simulink library "mbd_s32k1xx_ec_toolbox"  (Simulink 9.0)
(part 7 of 8)

      mask TypeOptions pinFtmCh5: None | PTD15: [FTM0_CH0 | FTM Channel] | PTB13: [FTM0_CH1 | FTM Channel] | PTC1: [FTM0_CH1 | FTM Channel] | PTD16: [FTM0_CH1 | FTM Channel] | PTC2: [FTM0_CH2 | FTM Channel] | PTD0: [FTM0_CH2 | FTM Channel] | PTC3: [FTM0_CH3 | FTM Channel] | PTD1: [FTM0_CH3 | FTM Channel] | PTB4: [FTM0_CH4 | FTM Channel] | PTB5: [FTM0_CH5 | FTM Channel] | PTE8: [FTM0_CH6 | FTM Channel] | PTE9: [FTM0_CH7 | FTM Channel] | PTB2: [FTM1_CH0 | FTM Channel] | PTC4: [FTM1_CH0 | FTM Channel] | PTA1: [FTM1_CH1 | FTM Channel] | PTB3: [FTM1_CH1 | FTM Channel] | PTC14: [FTM1_CH2 | FTM Channel] | PTC15: [FTM1_CH3 | FTM Channel] | PTA10: [FTM1_CH4 | FTM Channel] | PTA11: [FTM1_CH5 | FTM Channel] | PTA12: [FTM1_CH6 | FTM Channel] | PTA13: [FTM1_CH7 | FTM Channel] | PTC1: [FTM1_CH7 | FTM Channel] | PTD15: [FTM0_CH0 | FTM Channel] | PTB13: [FTM0_CH1 | FTM Channel] | PTC1: [FTM0_CH1 | FTM Channel] | PTD16: [FTM0_CH1 | FTM Channel] | PTC2: [FTM0_CH2 | FTM Channel] | PTD0: [FTM0_CH2 | FTM Channel] | PTC3: [FTM0_CH3 | FTM Channel] | PTD1: [FTM0_CH3 | FTM Channel] | PTB4: [FTM0_CH4 | FTM Channel] | PTB5: [FTM0_CH5 | FTM Channel] | PTE8: [FTM0_CH6 | FTM Channel] | PTE9: [FTM0_CH7 | FTM Channel] | PTB2: [FTM1_CH0 | FTM Channel] | PTC4: [FTM1_CH0 | FTM Channel] | PTA1: [FTM1_CH1 | FTM Channel] | PTB3: [FTM1_CH1 | FTM Channel] | PTC14: [FTM1_CH2 | FTM Channel] | PTC15: [FTM1_CH3 | FTM Channel] | PTA10: [FTM1_CH4 | FTM Channel] | PTA11: [FTM1_CH5 | FTM Channel] | PTA12: [FTM1_CH6 | FTM Channel] | PTA13: [FTM1_CH7 | FTM Channel] | PTC1: [FTM1_CH7 | FTM Channel] | PTD15: [FTM0_CH0 | FTM Channel] | PTB13: [FTM0_CH1 | FTM Channel] | PTC1: [FTM0_CH1 | FTM Channel] | PTD16: [FTM0_CH1 | FTM Channel] | PTC2: [FTM0_CH2 | FTM Channel] | PTD0: [FTM0_CH2 | FTM Channel] | PTC3: [FTM0_CH3 | FTM Channel] | PTD1: [FTM0_CH3 | FTM Channel] | PTB4: [FTM0_CH4 | FTM Channel] | PTB5: [FTM0_CH5 | FTM Channel] | PTE8: [FTM0_CH6 | FTM Channel] | PTE9: [FTM0_CH7 | FTM Channel] | PTB2: [FTM1_CH0 | FTM Channel] | PTC4: [FTM1_CH0 | FTM Channel] | PTA1: [FTM1_CH1 | FTM Channel] | PTB3: [FTM1_CH1 | FTM Channel] | PTC14: [FTM1_CH2 | FTM Channel] | PTC15: [FTM1_CH3 | FTM Channel] | PTA10: [FTM1_CH4 | FTM Channel] | PTA11: [FTM1_CH5 | FTM Channel] | PTA12: [FTM1_CH6 | FTM Channel] | PTA13: [FTM1_CH7 | FTM Channel] | PTC1: [FTM1_CH7 | FTM Channel] | PTC5: [FTM2_CH0 | FTM Channel] | PTD0: [FTM2_CH0 | FTM Channel] | PTD10: [FTM2_CH0 | FTM Channel] | PTA0: [FTM2_CH1 | FTM Channel] | PTD1: [FTM2_CH1 | FTM Channel] | PTD11: [FTM2_CH1 | FTM Channel] | PTD12: [FTM2_CH2 | FTM Channel] | PTE4: [FTM2_CH2 | FTM Channel] | PTD5: [FTM2_CH3 | FTM Channel] | PTE5: [FTM2_CH3 | FTM Channel] | PTD13: [FTM2_CH4 | FTM Channel] | PTE10: [FTM2_CH4 | FTM Channel] | PTD14: [FTM2_CH5 | FTM Channel] | PTE11: [FTM2_CH5 | FTM Channel] | PTC12: [FTM2_CH6 | FTM Channel] | PTE15: [FTM2_CH6 | FTM Channel] | PTC13: [FTM2_CH7 | FTM Channel] | PTE16: [FTM2_CH7 | FTM Channel] | PTA2: [FTM3_CH0 | FTM Channel] | PTB8: [FTM3_CH0 | FTM Channel] | PTA3: [FTM3_CH1 | FTM Channel] | PTB9: [FTM3_CH1 | FTM Channel] | PTB10: [FTM3_CH2 | FTM Channel] | PTC6: [FTM3_CH2 | FTM Channel] | PTB11: [FTM3_CH3 | FTM Channel] | PTC7: [FTM3_CH3 | FTM Channel] | PTC10: [FTM3_CH4 | FTM Channel] | PTD2: [FTM3_CH4 | FTM Channel] | PTC11: [FTM3_CH5 | FTM Channel] | PTD3: [FTM3_CH5 | FTM Channel] | PTC12: [FTM3_CH6 | FTM Channel] | PTE2: [FTM3_CH6 | FTM Channel] | PTC13: [FTM3_CH7 | FTM Channel] | PTE6: [FTM3_CH7 | FTM Channel] | PTD15: [FTM0_CH0 | FTM Channel] | PTB13: [FTM0_CH1 | FTM Channel] | PTC1: [FTM0_CH1 | FTM Channel] | PTD16: [FTM0_CH1 | FTM Channel] | PTC2: [FTM0_CH2 | FTM Channel] | PTD0: [FTM0_CH2 | FTM Channel] | PTC3: [FTM0_CH3 | FTM Channel] | PTD1: [FTM0_CH3 | FTM Channel] | PTB4: [FTM0_CH4 | FTM Channel] | PTB5: [FTM0_CH5 | FTM Channel] | PTE8: [FTM0_CH6 | FTM Channel] | PTE9: [FTM0_CH7 | FTM Channel] | PTB2: [FTM1_CH0 | FTM Channel] | PTC4: [FTM1_CH0 | FTM Channel] | PTA1: [FTM1_CH1 | FTM Channel] | PTB3: [FTM1_CH1 | FTM Channel] | PTC14: [FTM1_CH2 | FTM Channel] | PTC15: [FTM1_CH3 | FTM Channel] | PTA10: [FTM1_CH4 | FTM Channel] | PTA11: [FTM1_CH5 | FTM Channel] | PTA12: [FTM1_CH6 | FTM Channel] | PTA13: [FTM1_CH7 | FTM Channel] | PTC1: [FTM1_CH7 | FTM Channel] | PTC5: [FTM2_CH0 | FTM Channel] | PTD0: [FTM2_CH0 | FTM Channel] | PTD10: [FTM2_CH0 | FTM Channel] | PTA0: [FTM2_CH1 | FTM Channel] | PTD1: [FTM2_CH1 | FTM Channel] | PTD11: [FTM2_CH1 | FTM Channel] | PTD12: [FTM2_CH2 | FTM Channel] | PTE4: [FTM2_CH2 | FTM Channel] | PTD5: [FTM2_CH3 | FTM Channel] | PTE5: [FTM2_CH3 | FTM Channel] | PTD13: [FTM2_CH4 | FTM Channel] | PTE10: [FTM2_CH4 | FTM Channel] | PTD14: [FTM2_CH5 | FTM Channel] | PTE11: [FTM2_CH5 | FTM Channel] | PTC12: [FTM2_CH6 | FTM Channel] | PTE15: [FTM2_CH6 | FTM Channel] | PTC13: [FTM2_CH7 | FTM Channel] | PTE16: [FTM2_CH7 | FTM Channel] | PTA2: [FTM3_CH0 | FTM Channel] | PTB8: [FTM3_CH0 | FTM Channel] | PTA3: [FTM3_CH1 | FTM Channel] | PTB9: [FTM3_CH1 | FTM Channel] | PTB10: [FTM3_CH2 | FTM Channel] | PTC6: [FTM3_CH2 | FTM Channel] | PTB11: [FTM3_CH3 | FTM Channel] | PTC7: [FTM3_CH3 | FTM Channel] | PTC10: [FTM3_CH4 | FTM Channel] | PTD2: [FTM3_CH4 | FTM Channel] | PTC11: [FTM3_CH5 | FTM Channel] | PTD3: [FTM3_CH5 | FTM Channel] | PTC12: [FTM3_CH6 | FTM Channel] | PTE2: [FTM3_CH6 | FTM Channel] | PTC13: [FTM3_CH7 | FTM Channel] | PTE6: [FTM3_CH7 | FTM Channel] | PTD15: [FTM0_CH0 | FTM Channel] | PTB13: [FTM0_CH1 | FTM Channel] | PTC1: [FTM0_CH1 | FTM Channel] | PTD16: [FTM0_CH1 | FTM Channel] | PTC2: [FTM0_CH2 | FTM Channel] | PTD0: [FTM0_CH2 | FTM Channel] | PTC3: [FTM0_CH3 | FTM Channel] | PTD1: [FTM0_CH3 | FTM Channel] | PTB4: [FTM0_CH4 | FTM Channel] | PTB5: [FTM0_CH5 | FTM Channel] | PTE8: [FTM0_CH6 | FTM Channel] | PTE9: [FTM0_CH7 | FTM Channel] | PTB2: [FTM1_CH0 | FTM Channel] | PTC4: [FTM1_CH0 | FTM Channel] | PTA1: [FTM1_CH1 | FTM Channel] | PTB3: [FTM1_CH1 | FTM Channel] | PTC14: [FTM1_CH2 | FTM Channel] | PTC15: [FTM1_CH3 | FTM Channel] | PTA10: [FTM1_CH4 | FTM Channel] | PTA11: [FTM1_CH5 | FTM Channel] | PTA12: [FTM1_CH6 | FTM Channel] | PTA13: [FTM1_CH7 | FTM Channel] | PTC1: [FTM1_CH7 | FTM Channel] | PTC5: [FTM2_CH0 | FTM Channel] | PTD0: [FTM2_CH0 | FTM Channel] | PTD10: [FTM2_CH0 | FTM Channel] | PTA0: [FTM2_CH1 | FTM Channel] | PTD1: [FTM2_CH1 | FTM Channel] | PTD11: [FTM2_CH1 | FTM Channel] | PTD12: [FTM2_CH2 | FTM Channel] | PTE4: [FTM2_CH2 | FTM Channel] | PTD5: [FTM2_CH3 | FTM Channel] | PTE5: [FTM2_CH3 | FTM Channel] | PTD13: [FTM2_CH4 | FTM Channel] | PTE10: [FTM2_CH4 | FTM Channel] | PTD14: [FTM2_CH5 | FTM Channel] | PTE11: [FTM2_CH5 | FTM Channel] | PTC12: [FTM2_CH6 | FTM Channel] | PTE15: [FTM2_CH6 | FTM Channel] | PTC13: [FTM2_CH7 | FTM Channel] | PTE16: [FTM2_CH7 | FTM Channel] | PTA2: [FTM3_CH0 | FTM Channel] | PTB8: [FTM3_CH0 | FTM Channel] | PTA3: [FTM3_CH1 | FTM Channel] | PTB9: [FTM3_CH1 | FTM Channel] | PTB10: [FTM3_CH2 | FTM Channel] | PTC6: [FTM3_CH2 | FTM Channel] | PTB11: [FTM3_CH3 | FTM Channel] | PTC7: [FTM3_CH3 | FTM Channel] | PTC10: [FTM3_CH4 | FTM Channel] | PTD2: [FTM3_CH4 | FTM Channel] | PTC11: [FTM3_CH5 | FTM Channel] | PTD3: [FTM3_CH5 | FTM Channel] | PTC12: [FTM3_CH6 | FTM Channel] | PTE2: [FTM3_CH6 | FTM Channel] | PTC13: [FTM3_CH7 | FTM Channel] | PTE6: [FTM3_CH7 | FTM Channel] | PTE20: [FTM4_CH0 | FTM Channel] | PTE21: [FTM4_CH1 | FTM Channel] | PTC11: [FTM4_CH2 | FTM Channel] | PTE22: [FTM4_CH2 | FTM Channel] | PTE23: [FTM4_CH3 | FTM Channel] | PTC27: [FTM4_CH4 | FTM Channel] | PTE24: [FTM4_CH4 | FTM Channel] | PTB1: [FTM4_CH5 | FTM Channel] | PTE13: [FTM4_CH5 | FTM Channel] | PTE25: [FTM4_CH5 | FTM Channel] | PTB0: [FTM4_CH6 | FTM Channel] | PTC28: [FTM4_CH7 | FTM Channel] | PTA25: [FTM5_CH0 | FTM Channel] | PTC9: [FTM5_CH0 | FTM Channel] | PTA26: [FTM5_CH1 | FTM Channel] | PTC8: [FTM5_CH1 | FTM Channel] | PTA27: [FTM5_CH2 | FTM Channel] | PTC29: [FTM5_CH2 | FTM Channel] | PTA7: [FTM5_CH3 | FTM Channel] | PTA28: [FTM5_CH3 | FTM Channel] | PTA29: [FTM5_CH4 | FTM Channel] | PTC30: [FTM5_CH4 | FTM Channel] | PTA6: [FTM5_CH5 | FTM Channel] | PTA30: [FTM5_CH5 | FTM Channel] | PTA31: [FTM5_CH6 | FTM Channel] | PTC31: [FTM5_CH6 | FTM Channel] | PTB18: [FTM5_CH7 | FTM Channel] | PTD18: [FTM5_CH7 | FTM Channel] | PTD15: [FTM0_CH0 | FTM Channel] | PTB13: [FTM0_CH1 | FTM Channel] | PTC1: [FTM0_CH1 | FTM Channel] | PTD16: [FTM0_CH1 | FTM Channel] | PTC2: [FTM0_CH2 | FTM Channel] | PTD0: [FTM0_CH2 | FTM Channel] | PTC3: [FTM0_CH3 | FTM Channel] | PTD1: [FTM0_CH3 | FTM Channel] | PTB4: [FTM0_CH4 | FTM Channel] | PTB5: [FTM0_CH5 | FTM Channel] | PTE8: [FTM0_CH6 | FTM Channel] | PTE9: [FTM0_CH7 | FTM Channel] | PTB2: [FTM1_CH0 | FTM Channel] | PTC4: [FTM1_CH0 | FTM Channel] | PTA1: [FTM1_CH1 | FTM Channel] | PTB3: [FTM1_CH1 | FTM Channel] | PTC14: [FTM1_CH2 | FTM Channel] | PTC15: [FTM1_CH3 | FTM Channel] | PTA10: [FTM1_CH4 | FTM Channel] | PTA11: [FTM1_CH5 | FTM Channel] | PTA12: [FTM1_CH6 | FTM Channel] | PTA13: [FTM1_CH7 | FTM Channel] | PTC1: [FTM1_CH7 | FTM Channel] | PTC5: [FTM2_CH0 | FTM Channel] | PTD0: [FTM2_CH0 | FTM Channel] | PTD10: [FTM2_CH0 | FTM Channel] | PTA0: [FTM2_CH1 | FTM Channel] | PTD1: [FTM2_CH1 | FTM Channel] | PTD11: [FTM2_CH1 | FTM Channel] | PTD12: [FTM2_CH2 | FTM Channel] | PTE4: [FTM2_CH2 | FTM Channel] | PTD5: [FTM2_CH3 | FTM Channel] | PTE5: [FTM2_CH3 | FTM Channel] | PTD13: [FTM2_CH4 | FTM Channel] | PTE10: [FTM2_CH4 | FTM Channel] | PTD14: [FTM2_CH5 | FTM Channel] | PTE11: [FTM2_CH5 | FTM Channel] | PTC12: [FTM2_CH6 | FTM Channel] | PTE15: [FTM2_CH6 | FTM Channel] | PTC13: [FTM2_CH7 | FTM Channel] | PTE16: [FTM2_CH7 | FTM Channel] | PTA2: [FTM3_CH0 | FTM Channel] | PTB8: [FTM3_CH0 | FTM Channel] | PTA3: [FTM3_CH1 | FTM Channel] | PTB9: [FTM3_CH1 | FTM Channel] | PTB10: [FTM3_CH2 | FTM Channel] | PTC6: [FTM3_CH2 | FTM Channel] | PTB11: [FTM3_CH3 | FTM Channel] | PTC7: [FTM3_CH3 | FTM Channel] | PTC10: [FTM3_CH4 | FTM Channel] | PTD2: [FTM3_CH4 | FTM Channel] | PTC11: [FTM3_CH5 | FTM Channel] | PTD3: [FTM3_CH5 | FTM Channel] | PTC12: [FTM3_CH6 | FTM Channel] | PTE2: [FTM3_CH6 | FTM Channel] | PTC13: [FTM3_CH7 | FTM Channel] | PTE6: [FTM3_CH7 | FTM Channel] | PTE20: [FTM4_CH0 | FTM Channel] | PTE21: [FTM4_CH1 | FTM Channel] | PTC11: [FTM4_CH2 | FTM Channel] | PTE22: [FTM4_CH2 | FTM Channel] | PTE23: [FTM4_CH3 | FTM Channel] | PTC27: [FTM4_CH4 | FTM Channel] | PTE24: [FTM4_CH4 | FTM Channel] | PTB1: [FTM4_CH5 | FTM Channel] | PTE13: [FTM4_CH5 | FTM Channel] | PTE25: [FTM4_CH5 | FTM Channel] | PTB0: [FTM4_CH6 | FTM Channel] | PTC28: [FTM4_CH7 | FTM Channel] | PTA25: [FTM5_CH0 | FTM Channel] | PTC9: [FTM5_CH0 | FTM Channel] | PTA26: [FTM5_CH1 | FTM Channel] | PTC8: [FTM5_CH1 | FTM Channel] | PTA27: [FTM5_CH2 | FTM Channel] | PTC29: [FTM5_CH2 | FTM Channel] | PTA7: [FTM5_CH3 | FTM Channel] | PTA28: [FTM5_CH3 | FTM Channel] | PTA29: [FTM5_CH4 | FTM Channel] | PTC30: [FTM5_CH4 | FTM Channel] | PTA6: [FTM5_CH5 | FTM Channel] | PTA30: [FTM5_CH5 | FTM Channel] | PTA31: [FTM5_CH6 | FTM Channel] | PTC31: [FTM5_CH6 | FTM Channel] | PTB18: [FTM5_CH7 | FTM Channel] | PTD18: [FTM5_CH7 | FTM Channel] | PTA18: [FTM6_CH0 | FTM Channel] | PTB20: [FTM6_CH0 | FTM Channel] | PTD19: [FTM6_CH0 | FTM Channel] | PTB21: [FTM6_CH1 | FTM Channel] | PTD20: [FTM6_CH1 | FTM Channel] | PTB22: [FTM6_CH2 | FTM Channel] | PTD21: [FTM6_CH2 | FTM Channel] | PTB23: [FTM6_CH3 | FTM Channel] | PTD22: [FTM6_CH3 | FTM Channel] | PTB24: [FTM6_CH4 | FTM Channel] | PTD23: [FTM6_CH4 | FTM Channel] | PTB25: [FTM6_CH5 | FTM Channel] | PTD24: [FTM6_CH5 | FTM Channel] | PTB26: [FTM6_CH6 | FTM Channel] | PTD25: [FTM6_CH6 | FTM Channel] | PTB27: [FTM6_CH7 | FTM Channel] | PTD26: [FTM6_CH7 | FTM Channel] | PTB28: [FTM7_CH0 | FTM Channel] | PTD27: [FTM7_CH0 | FTM Channel] | PTB29: [FTM7_CH1 | FTM Channel] | PTD28: [FTM7_CH1 | FTM Channel] | PTB30: [FTM7_CH2 | FTM Channel] | PTD29: [FTM7_CH2 | FTM Channel] | PTB31: [FTM7_CH3 | FTM Channel] | PTD30: [FTM7_CH3 | FTM Channel] | PTC18: [FTM7_CH4 | FTM Channel] | PTD31: [FTM7_CH4 | FTM Channel] | PTC19: [FTM7_CH5 | FTM Channel] | PTE17: [FTM7_CH5 | FTM Channel] | PTC20: [FTM7_CH6 | FTM Channel] | PTE18: [FTM7_CH6 | FTM Channel] | PTC21: [FTM7_CH7 | FTM Channel] | PTE19: [FTM7_CH7 | FTM Channel]
      mask TypeOptions pinPolCh4: Active Low | Active High
      mask TypeOptions pinPolCh5: Active Low | Active High
      mask TypeOptions outputComplem4: Main duplicated | Main inverted
      mask TypeOptions outputLevel4: Low | High
      mask TypeOptions outputLevel5: Low | High
      mask TypeOptions pinFtmCh6: PTD15: [FTM0_CH0 | FTM Channel] | PTB13: [FTM0_CH1 | FTM Channel] | PTC1: [FTM0_CH1 | FTM Channel] | PTD16: [FTM0_CH1 | FTM Channel] | PTC2: [FTM0_CH2 | FTM Channel] | PTD0: [FTM0_CH2 | FTM Channel] | PTC3: [FTM0_CH3 | FTM Channel] | PTD1: [FTM0_CH3 | FTM Channel] | PTB4: [FTM0_CH4 | FTM Channel] | PTB5: [FTM0_CH5 | FTM Channel] | PTE8: [FTM0_CH6 | FTM Channel] | PTE9: [FTM0_CH7 | FTM Channel] | PTB2: [FTM1_CH0 | FTM Channel] | PTC4: [FTM1_CH0 | FTM Channel] | PTA1: [FTM1_CH1 | FTM Channel] | PTB3: [FTM1_CH1 | FTM Channel] | PTC14: [FTM1_CH2 | FTM Channel] | PTC15: [FTM1_CH3 | FTM Channel] | PTA10: [FTM1_CH4 | FTM Channel] | PTA11: [FTM1_CH5 | FTM Channel] | PTA12: [FTM1_CH6 | FTM Channel] | PTA13: [FTM1_CH7 | FTM Channel] | PTC1: [FTM1_CH7 | FTM Channel] | PTD15: [FTM0_CH0 | FTM Channel] | PTB13: [FTM0_CH1 | FTM Channel] | PTC1: [FTM0_CH1 | FTM Channel] | PTD16: [FTM0_CH1 | FTM Channel] | PTC2: [FTM0_CH2 | FTM Channel] | PTD0: [FTM0_CH2 | FTM Channel] | PTC3: [FTM0_CH3 | FTM Channel] | PTD1: [FTM0_CH3 | FTM Channel] | PTB4: [FTM0_CH4 | FTM Channel] | PTB5: [FTM0_CH5 | FTM Channel] | PTE8: [FTM0_CH6 | FTM Channel] | PTE9: [FTM0_CH7 | FTM Channel] | PTB2: [FTM1_CH0 | FTM Channel] | PTC4: [FTM1_CH0 | FTM Channel] | PTA1: [FTM1_CH1 | FTM Channel] | PTB3: [FTM1_CH1 | FTM Channel] | PTC14: [FTM1_CH2 | FTM Channel] | PTC15: [FTM1_CH3 | FTM Channel] | PTA10: [FTM1_CH4 | FTM Channel] | PTA11: [FTM1_CH5 | FTM Channel] | PTA12: [FTM1_CH6 | FTM Channel] | PTA13: [FTM1_CH7 | FTM Channel] | PTC1: [FTM1_CH7 | FTM Channel] | PTD15: [FTM0_CH0 | FTM Channel] | PTB13: [FTM0_CH1 | FTM Channel] | PTC1: [FTM0_CH1 | FTM Channel] | PTD16: [FTM0_CH1 | FTM Channel] | PTC2: [FTM0_CH2 | FTM Channel] | PTD0: [FTM0_CH2 | FTM Channel] | PTC3: [FTM0_CH3 | FTM Channel] | PTD1: [FTM0_CH3 | FTM Channel] | PTB4: [FTM0_CH4 | FTM Channel] | PTB5: [FTM0_CH5 | FTM Channel] | PTE8: [FTM0_CH6 | FTM Channel] | PTE9: [FTM0_CH7 | FTM Channel] | PTB2: [FTM1_CH0 | FTM Channel] | PTC4: [FTM1_CH0 | FTM Channel] | PTA1: [FTM1_CH1 | FTM Channel] | PTB3: [FTM1_CH1 | FTM Channel] | PTC14: [FTM1_CH2 | FTM Channel] | PTC15: [FTM1_CH3 | FTM Channel] | PTA10: [FTM1_CH4 | FTM Channel] | PTA11: [FTM1_CH5 | FTM Channel] | PTA12: [FTM1_CH6 | FTM Channel] | PTA13: [FTM1_CH7 | FTM Channel] | PTC1: [FTM1_CH7 | FTM Channel] | PTC5: [FTM2_CH0 | FTM Channel] | PTD0: [FTM2_CH0 | FTM Channel] | PTD10: [FTM2_CH0 | FTM Channel] | PTA0: [FTM2_CH1 | FTM Channel] | PTD1: [FTM2_CH1 | FTM Channel] | PTD11: [FTM2_CH1 | FTM Channel] | PTD12: [FTM2_CH2 | FTM Channel] | PTE4: [FTM2_CH2 | FTM Channel] | PTD5: [FTM2_CH3 | FTM Channel] | PTE5: [FTM2_CH3 | FTM Channel] | PTD13: [FTM2_CH4 | FTM Channel] | PTE10: [FTM2_CH4 | FTM Channel] | PTD14: [FTM2_CH5 | FTM Channel] | PTE11: [FTM2_CH5 | FTM Channel] | PTC12: [FTM2_CH6 | FTM Channel] | PTE15: [FTM2_CH6 | FTM Channel] | PTC13: [FTM2_CH7 | FTM Channel] | PTE16: [FTM2_CH7 | FTM Channel] | PTA2: [FTM3_CH0 | FTM Channel] | PTB8: [FTM3_CH0 | FTM Channel] | PTA3: [FTM3_CH1 | FTM Channel] | PTB9: [FTM3_CH1 | FTM Channel] | PTB10: [FTM3_CH2 | FTM Channel] | PTC6: [FTM3_CH2 | FTM Channel] | PTB11: [FTM3_CH3 | FTM Channel] | PTC7: [FTM3_CH3 | FTM Channel] | PTC10: [FTM3_CH4 | FTM Channel] | PTD2: [FTM3_CH4 | FTM Channel] | PTC11: [FTM3_CH5 | FTM Channel] | PTD3: [FTM3_CH5 | FTM Channel] | PTC12: [FTM3_CH6 | FTM Channel] | PTE2: [FTM3_CH6 | FTM Channel] | PTC13: [FTM3_CH7 | FTM Channel] | PTE6: [FTM3_CH7 | FTM Channel] | PTD15: [FTM0_CH0 | FTM Channel] | PTB13: [FTM0_CH1 | FTM Channel] | PTC1: [FTM0_CH1 | FTM Channel] | PTD16: [FTM0_CH1 | FTM Channel] | PTC2: [FTM0_CH2 | FTM Channel] | PTD0: [FTM0_CH2 | FTM Channel] | PTC3: [FTM0_CH3 | FTM Channel] | PTD1: [FTM0_CH3 | FTM Channel] | PTB4: [FTM0_CH4 | FTM Channel] | PTB5: [FTM0_CH5 | FTM Channel] | PTE8: [FTM0_CH6 | FTM Channel] | PTE9: [FTM0_CH7 | FTM Channel] | PTB2: [FTM1_CH0 | FTM Channel] | PTC4: [FTM1_CH0 | FTM Channel] | PTA1: [FTM1_CH1 | FTM Channel] | PTB3: [FTM1_CH1 | FTM Channel] | PTC14: [FTM1_CH2 | FTM Channel] | PTC15: [FTM1_CH3 | FTM Channel] | PTA10: [FTM1_CH4 | FTM Channel] | PTA11: [FTM1_CH5 | FTM Channel] | PTA12: [FTM1_CH6 | FTM Channel] | PTA13: [FTM1_CH7 | FTM Channel] | PTC1: [FTM1_CH7 | FTM Channel] | PTC5: [FTM2_CH0 | FTM Channel] | PTD0: [FTM2_CH0 | FTM Channel] | PTD10: [FTM2_CH0 | FTM Channel] | PTA0: [FTM2_CH1 | FTM Channel] | PTD1: [FTM2_CH1 | FTM Channel] | PTD11: [FTM2_CH1 | FTM Channel] | PTD12: [FTM2_CH2 | FTM Channel] | PTE4: [FTM2_CH2 | FTM Channel] | PTD5: [FTM2_CH3 | FTM Channel] | PTE5: [FTM2_CH3 | FTM Channel] | PTD13: [FTM2_CH4 | FTM Channel] | PTE10: [FTM2_CH4 | FTM Channel] | PTD14: [FTM2_CH5 | FTM Channel] | PTE11: [FTM2_CH5 | FTM Channel] | PTC12: [FTM2_CH6 | FTM Channel] | PTE15: [FTM2_CH6 | FTM Channel] | PTC13: [FTM2_CH7 | FTM Channel] | PTE16: [FTM2_CH7 | FTM Channel] | PTA2: [FTM3_CH0 | FTM Channel] | PTB8: [FTM3_CH0 | FTM Channel] | PTA3: [FTM3_CH1 | FTM Channel] | PTB9: [FTM3_CH1 | FTM Channel] | PTB10: [FTM3_CH2 | FTM Channel] | PTC6: [FTM3_CH2 | FTM Channel] | PTB11: [FTM3_CH3 | FTM Channel] | PTC7: [FTM3_CH3 | FTM Channel] | PTC10: [FTM3_CH4 | FTM Channel] | PTD2: [FTM3_CH4 | FTM Channel] | PTC11: [FTM3_CH5 | FTM Channel] | PTD3: [FTM3_CH5 | FTM Channel] | PTC12: [FTM3_CH6 | FTM Channel] | PTE2: [FTM3_CH6 | FTM Channel] | PTC13: [FTM3_CH7 | FTM Channel] | PTE6: [FTM3_CH7 | FTM Channel] | PTD15: [FTM0_CH0 | FTM Channel] | PTB13: [FTM0_CH1 | FTM Channel] | PTC1: [FTM0_CH1 | FTM Channel] | PTD16: [FTM0_CH1 | FTM Channel] | PTC2: [FTM0_CH2 | FTM Channel] | PTD0: [FTM0_CH2 | FTM Channel] | PTC3: [FTM0_CH3 | FTM Channel] | PTD1: [FTM0_CH3 | FTM Channel] | PTB4: [FTM0_CH4 | FTM Channel] | PTB5: [FTM0_CH5 | FTM Channel] | PTE8: [FTM0_CH6 | FTM Channel] | PTE9: [FTM0_CH7 | FTM Channel] | PTB2: [FTM1_CH0 | FTM Channel] | PTC4: [FTM1_CH0 | FTM Channel] | PTA1: [FTM1_CH1 | FTM Channel] | PTB3: [FTM1_CH1 | FTM Channel] | PTC14: [FTM1_CH2 | FTM Channel] | PTC15: [FTM1_CH3 | FTM Channel] | PTA10: [FTM1_CH4 | FTM Channel] | PTA11: [FTM1_CH5 | FTM Channel] | PTA12: [FTM1_CH6 | FTM Channel] | PTA13: [FTM1_CH7 | FTM Channel] | PTC1: [FTM1_CH7 | FTM Channel] | PTC5: [FTM2_CH0 | FTM Channel] | PTD0: [FTM2_CH0 | FTM Channel] | PTD10: [FTM2_CH0 | FTM Channel] | PTA0: [FTM2_CH1 | FTM Channel] | PTD1: [FTM2_CH1 | FTM Channel] | PTD11: [FTM2_CH1 | FTM Channel] | PTD12: [FTM2_CH2 | FTM Channel] | PTE4: [FTM2_CH2 | FTM Channel] | PTD5: [FTM2_CH3 | FTM Channel] | PTE5: [FTM2_CH3 | FTM Channel] | PTD13: [FTM2_CH4 | FTM Channel] | PTE10: [FTM2_CH4 | FTM Channel] | PTD14: [FTM2_CH5 | FTM Channel] | PTE11: [FTM2_CH5 | FTM Channel] | PTC12: [FTM2_CH6 | FTM Channel] | PTE15: [FTM2_CH6 | FTM Channel] | PTC13: [FTM2_CH7 | FTM Channel] | PTE16: [FTM2_CH7 | FTM Channel] | PTA2: [FTM3_CH0 | FTM Channel] | PTB8: [FTM3_CH0 | FTM Channel] | PTA3: [FTM3_CH1 | FTM Channel] | PTB9: [FTM3_CH1 | FTM Channel] | PTB10: [FTM3_CH2 | FTM Channel] | PTC6: [FTM3_CH2 | FTM Channel] | PTB11: [FTM3_CH3 | FTM Channel] | PTC7: [FTM3_CH3 | FTM Channel] | PTC10: [FTM3_CH4 | FTM Channel] | PTD2: [FTM3_CH4 | FTM Channel] | PTC11: [FTM3_CH5 | FTM Channel] | PTD3: [FTM3_CH5 | FTM Channel] | PTC12: [FTM3_CH6 | FTM Channel] | PTE2: [FTM3_CH6 | FTM Channel] | PTC13: [FTM3_CH7 | FTM Channel] | PTE6: [FTM3_CH7 | FTM Channel] | PTE20: [FTM4_CH0 | FTM Channel] | PTE21: [FTM4_CH1 | FTM Channel] | PTC11: [FTM4_CH2 | FTM Channel] | PTE22: [FTM4_CH2 | FTM Channel] | PTE23: [FTM4_CH3 | FTM Channel] | PTC27: [FTM4_CH4 | FTM Channel] | PTE24: [FTM4_CH4 | FTM Channel] | PTB1: [FTM4_CH5 | FTM Channel] | PTE13: [FTM4_CH5 | FTM Channel] | PTE25: [FTM4_CH5 | FTM Channel] | PTB0: [FTM4_CH6 | FTM Channel] | PTC28: [FTM4_CH7 | FTM Channel] | PTA25: [FTM5_CH0 | FTM Channel] | PTC9: [FTM5_CH0 | FTM Channel] | PTA26: [FTM5_CH1 | FTM Channel] | PTC8: [FTM5_CH1 | FTM Channel] | PTA27: [FTM5_CH2 | FTM Channel] | PTC29: [FTM5_CH2 | FTM Channel] | PTA7: [FTM5_CH3 | FTM Channel] | PTA28: [FTM5_CH3 | FTM Channel] | PTA29: [FTM5_CH4 | FTM Channel] | PTC30: [FTM5_CH4 | FTM Channel] | PTA6: [FTM5_CH5 | FTM Channel] | PTA30: [FTM5_CH5 | FTM Channel] | PTA31: [FTM5_CH6 | FTM Channel] | PTC31: [FTM5_CH6 | FTM Channel] | PTB18: [FTM5_CH7 | FTM Channel] | PTD18: [FTM5_CH7 | FTM Channel] | PTD15: [FTM0_CH0 | FTM Channel] | PTB13: [FTM0_CH1 | FTM Channel] | PTC1: [FTM0_CH1 | FTM Channel] | PTD16: [FTM0_CH1 | FTM Channel] | PTC2: [FTM0_CH2 | FTM Channel] | PTD0: [FTM0_CH2 | FTM Channel] | PTC3: [FTM0_CH3 | FTM Channel] | PTD1: [FTM0_CH3 | FTM Channel] | PTB4: [FTM0_CH4 | FTM Channel] | PTB5: [FTM0_CH5 | FTM Channel] | PTE8: [FTM0_CH6 | FTM Channel] | PTE9: [FTM0_CH7 | FTM Channel] | PTB2: [FTM1_CH0 | FTM Channel] | PTC4: [FTM1_CH0 | FTM Channel] | PTA1: [FTM1_CH1 | FTM Channel] | PTB3: [FTM1_CH1 | FTM Channel] | PTC14: [FTM1_CH2 | FTM Channel] | PTC15: [FTM1_CH3 | FTM Channel] | PTA10: [FTM1_CH4 | FTM Channel] | PTA11: [FTM1_CH5 | FTM Channel] | PTA12: [FTM1_CH6 | FTM Channel] | PTA13: [FTM1_CH7 | FTM Channel] | PTC1: [FTM1_CH7 | FTM Channel] | PTC5: [FTM2_CH0 | FTM Channel] | PTD0: [FTM2_CH0 | FTM Channel] | PTD10: [FTM2_CH0 | FTM Channel] | PTA0: [FTM2_CH1 | FTM Channel] | PTD1: [FTM2_CH1 | FTM Channel] | PTD11: [FTM2_CH1 | FTM Channel] | PTD12: [FTM2_CH2 | FTM Channel] | PTE4: [FTM2_CH2 | FTM Channel] | PTD5: [FTM2_CH3 | FTM Channel] | PTE5: [FTM2_CH3 | FTM Channel] | PTD13: [FTM2_CH4 | FTM Channel] | PTE10: [FTM2_CH4 | FTM Channel] | PTD14: [FTM2_CH5 | FTM Channel] | PTE11: [FTM2_CH5 | FTM Channel] | PTC12: [FTM2_CH6 | FTM Channel] | PTE15: [FTM2_CH6 | FTM Channel] | PTC13: [FTM2_CH7 | FTM Channel] | PTE16: [FTM2_CH7 | FTM Channel] | PTA2: [FTM3_CH0 | FTM Channel] | PTB8: [FTM3_CH0 | FTM Channel] | PTA3: [FTM3_CH1 | FTM Channel] | PTB9: [FTM3_CH1 | FTM Channel] | PTB10: [FTM3_CH2 | FTM Channel] | PTC6: [FTM3_CH2 | FTM Channel] | PTB11: [FTM3_CH3 | FTM Channel] | PTC7: [FTM3_CH3 | FTM Channel] | PTC10: [FTM3_CH4 | FTM Channel] | PTD2: [FTM3_CH4 | FTM Channel] | PTC11: [FTM3_CH5 | FTM Channel] | PTD3: [FTM3_CH5 | FTM Channel] | PTC12: [FTM3_CH6 | FTM Channel] | PTE2: [FTM3_CH6 | FTM Channel] | PTC13: [FTM3_CH7 | FTM Channel] | PTE6: [FTM3_CH7 | FTM Channel] | PTE20: [FTM4_CH0 | FTM Channel] | PTE21: [FTM4_CH1 | FTM Channel] | PTC11: [FTM4_CH2 | FTM Channel] | PTE22: [FTM4_CH2 | FTM Channel] | PTE23: [FTM4_CH3 | FTM Channel] | PTC27: [FTM4_CH4 | FTM Channel] | PTE24: [FTM4_CH4 | FTM Channel] | PTB1: [FTM4_CH5 | FTM Channel] | PTE13: [FTM4_CH5 | FTM Channel] | PTE25: [FTM4_CH5 | FTM Channel] | PTB0: [FTM4_CH6 | FTM Channel] | PTC28: [FTM4_CH7 | FTM Channel] | PTA25: [FTM5_CH0 | FTM Channel] | PTC9: [FTM5_CH0 | FTM Channel] | PTA26: [FTM5_CH1 | FTM Channel] | PTC8: [FTM5_CH1 | FTM Channel] | PTA27: [FTM5_CH2 | FTM Channel] | PTC29: [FTM5_CH2 | FTM Channel] | PTA7: [FTM5_CH3 | FTM Channel] | PTA28: [FTM5_CH3 | FTM Channel] | PTA29: [FTM5_CH4 | FTM Channel] | PTC30: [FTM5_CH4 | FTM Channel] | PTA6: [FTM5_CH5 | FTM Channel] | PTA30: [FTM5_CH5 | FTM Channel] | PTA31: [FTM5_CH6 | FTM Channel] | PTC31: [FTM5_CH6 | FTM Channel] | PTB18: [FTM5_CH7 | FTM Channel] | PTD18: [FTM5_CH7 | FTM Channel] | PTA18: [FTM6_CH0 | FTM Channel] | PTB20: [FTM6_CH0 | FTM Channel] | PTD19: [FTM6_CH0 | FTM Channel] | PTB21: [FTM6_CH1 | FTM Channel] | PTD20: [FTM6_CH1 | FTM Channel] | PTB22: [FTM6_CH2 | FTM Channel] | PTD21: [FTM6_CH2 | FTM Channel] | PTB23: [FTM6_CH3 | FTM Channel] | PTD22: [FTM6_CH3 | FTM Channel] | PTB24: [FTM6_CH4 | FTM Channel] | PTD23: [FTM6_CH4 | FTM Channel] | PTB25: [FTM6_CH5 | FTM Channel] | PTD24: [FTM6_CH5 | FTM Channel] | PTB26: [FTM6_CH6 | FTM Channel] | PTD25: [FTM6_CH6 | FTM Channel] | PTB27: [FTM6_CH7 | FTM Channel] | PTD26: [FTM6_CH7 | FTM Channel] | PTB28: [FTM7_CH0 | FTM Channel] | PTD27: [FTM7_CH0 | FTM Channel] | PTB29: [FTM7_CH1 | FTM Channel] | PTD28: [FTM7_CH1 | FTM Channel] | PTB30: [FTM7_CH2 | FTM Channel] | PTD29: [FTM7_CH2 | FTM Channel] | PTB31: [FTM7_CH3 | FTM Channel] | PTD30: [FTM7_CH3 | FTM Channel] | PTC18: [FTM7_CH4 | FTM Channel] | PTD31: [FTM7_CH4 | FTM Channel] | PTC19: [FTM7_CH5 | FTM Channel] | PTE17: [FTM7_CH5 | FTM Channel] | PTC20: [FTM7_CH6 | FTM Channel] | PTE18: [FTM7_CH6 | FTM Channel] | PTC21: [FTM7_CH7 | FTM Channel] | PTE19: [FTM7_CH7 | FTM Channel]
      mask TypeOptions pinFtmCh7: None | PTD15: [FTM0_CH0 | FTM Channel] | PTB13: [FTM0_CH1 | FTM Channel] | PTC1: [FTM0_CH1 | FTM Channel] | PTD16: [FTM0_CH1 | FTM Channel] | PTC2: [FTM0_CH2 | FTM Channel] | PTD0: [FTM0_CH2 | FTM Channel] | PTC3: [FTM0_CH3 | FTM Channel] | PTD1: [FTM0_CH3 | FTM Channel] | PTB4: [FTM0_CH4 | FTM Channel] | PTB5: [FTM0_CH5 | FTM Channel] | PTE8: [FTM0_CH6 | FTM Channel] | PTE9: [FTM0_CH7 | FTM Channel] | PTB2: [FTM1_CH0 | FTM Channel] | PTC4: [FTM1_CH0 | FTM Channel] | PTA1: [FTM1_CH1 | FTM Channel] | PTB3: [FTM1_CH1 | FTM Channel] | PTC14: [FTM1_CH2 | FTM Channel] | PTC15: [FTM1_CH3 | FTM Channel] | PTA10: [FTM1_CH4 | FTM Channel] | PTA11: [FTM1_CH5 | FTM Channel] | PTA12: [FTM1_CH6 | FTM Channel] | PTA13: [FTM1_CH7 | FTM Channel] | PTC1: [FTM1_CH7 | FTM Channel] | PTD15: [FTM0_CH0 | FTM Channel] | PTB13: [FTM0_CH1 | FTM Channel] | PTC1: [FTM0_CH1 | FTM Channel] | PTD16: [FTM0_CH1 | FTM Channel] | PTC2: [FTM0_CH2 | FTM Channel] | PTD0: [FTM0_CH2 | FTM Channel] | PTC3: [FTM0_CH3 | FTM Channel] | PTD1: [FTM0_CH3 | FTM Channel] | PTB4: [FTM0_CH4 | FTM Channel] | PTB5: [FTM0_CH5 | FTM Channel] | PTE8: [FTM0_CH6 | FTM Channel] | PTE9: [FTM0_CH7 | FTM Channel] | PTB2: [FTM1_CH0 | FTM Channel] | PTC4: [FTM1_CH0 | FTM Channel] | PTA1: [FTM1_CH1 | FTM Channel] | PTB3: [FTM1_CH1 | FTM Channel] | PTC14: [FTM1_CH2 | FTM Channel] | PTC15: [FTM1_CH3 | FTM Channel] | PTA10: [FTM1_CH4 | FTM Channel] | PTA11: [FTM1_CH5 | FTM Channel] | PTA12: [FTM1_CH6 | FTM Channel] | PTA13: [FTM1_CH7 | FTM Channel] | PTC1: [FTM1_CH7 | FTM Channel] | PTD15: [FTM0_CH0 | FTM Channel] | PTB13: [FTM0_CH1 | FTM Channel] | PTC1: [FTM0_CH1 | FTM Channel] | PTD16: [FTM0_CH1 | FTM Channel] | PTC2: [FTM0_CH2 | FTM Channel] | PTD0: [FTM0_CH2 | FTM Channel] | PTC3: [FTM0_CH3 | FTM Channel] | PTD1: [FTM0_CH3 | FTM Channel] | PTB4: [FTM0_CH4 | FTM Channel] | PTB5: [FTM0_CH5 | FTM Channel] | PTE8: [FTM0_CH6 | FTM Channel] | PTE9: [FTM0_CH7 | FTM Channel] | PTB2: [FTM1_CH0 | FTM Channel] | PTC4: [FTM1_CH0 | FTM Channel] | PTA1: [FTM1_CH1 | FTM Channel] | PTB3: [FTM1_CH1 | FTM Channel] | PTC14: [FTM1_CH2 | FTM Channel] | PTC15: [FTM1_CH3 | FTM Channel] | PTA10: [FTM1_CH4 | FTM Channel] | PTA11: [FTM1_CH5 | FTM Channel] | PTA12: [FTM1_CH6 | FTM Channel] | PTA13: [FTM1_CH7 | FTM Channel] | PTC1: [FTM1_CH7 | FTM Channel] | PTC5: [FTM2_CH0 | FTM Channel] | PTD0: [FTM2_CH0 | FTM Channel] | PTD10: [FTM2_CH0 | FTM Channel] | PTA0: [FTM2_CH1 | FTM Channel] | PTD1: [FTM2_CH1 | FTM Channel] | PTD11: [FTM2_CH1 | FTM Channel] | PTD12: [FTM2_CH2 | FTM Channel] | PTE4: [FTM2_CH2 | FTM Channel] | PTD5: [FTM2_CH3 | FTM Channel] | PTE5: [FTM2_CH3 | FTM Channel] | PTD13: [FTM2_CH4 | FTM Channel] | PTE10: [FTM2_CH4 | FTM Channel] | PTD14: [FTM2_CH5 | FTM Channel] | PTE11: [FTM2_CH5 | FTM Channel] | PTC12: [FTM2_CH6 | FTM Channel] | PTE15: [FTM2_CH6 | FTM Channel] | PTC13: [FTM2_CH7 | FTM Channel] | PTE16: [FTM2_CH7 | FTM Channel] | PTA2: [FTM3_CH0 | FTM Channel] | PTB8: [FTM3_CH0 | FTM Channel] | PTA3: [FTM3_CH1 | FTM Channel] | PTB9: [FTM3_CH1 | FTM Channel] | PTB10: [FTM3_CH2 | FTM Channel] | PTC6: [FTM3_CH2 | FTM Channel] | PTB11: [FTM3_CH3 | FTM Channel] | PTC7: [FTM3_CH3 | FTM Channel] | PTC10: [FTM3_CH4 | FTM Channel] | PTD2: [FTM3_CH4 | FTM Channel] | PTC11: [FTM3_CH5 | FTM Channel] | PTD3: [FTM3_CH5 | FTM Channel] | PTC12: [FTM3_CH6 | FTM Channel] | PTE2: [FTM3_CH6 | FTM Channel] | PTC13: [FTM3_CH7 | FTM Channel] | PTE6: [FTM3_CH7 | FTM Channel] | PTD15: [FTM0_CH0 | FTM Channel] | PTB13: [FTM0_CH1 | FTM Channel] | PTC1: [FTM0_CH1 | FTM Channel] | PTD16: [FTM0_CH1 | FTM Channel] | PTC2: [FTM0_CH2 | FTM Channel] | PTD0: [FTM0_CH2 | FTM Channel] | PTC3: [FTM0_CH3 | FTM Channel] | PTD1: [FTM0_CH3 | FTM Channel] | PTB4: [FTM0_CH4 | FTM Channel] | PTB5: [FTM0_CH5 | FTM Channel] | PTE8: [FTM0_CH6 | FTM Channel] | PTE9: [FTM0_CH7 | FTM Channel] | PTB2: [FTM1_CH0 | FTM Channel] | PTC4: [FTM1_CH0 | FTM Channel] | PTA1: [FTM1_CH1 | FTM Channel] | PTB3: [FTM1_CH1 | FTM Channel] | PTC14: [FTM1_CH2 | FTM Channel] | PTC15: [FTM1_CH3 | FTM Channel] | PTA10: [FTM1_CH4 | FTM Channel] | PTA11: [FTM1_CH5 | FTM Channel] | PTA12: [FTM1_CH6 | FTM Channel] | PTA13: [FTM1_CH7 | FTM Channel] | PTC1: [FTM1_CH7 | FTM Channel] | PTC5: [FTM2_CH0 | FTM Channel] | PTD0: [FTM2_CH0 | FTM Channel] | PTD10: [FTM2_CH0 | FTM Channel] | PTA0: [FTM2_CH1 | FTM Channel] | PTD1: [FTM2_CH1 | FTM Channel] | PTD11: [FTM2_CH1 | FTM Channel] | PTD12: [FTM2_CH2 | FTM Channel] | PTE4: [FTM2_CH2 | FTM Channel] | PTD5: [FTM2_CH3 | FTM Channel] | PTE5: [FTM2_CH3 | FTM Channel] | PTD13: [FTM2_CH4 | FTM Channel] | PTE10: [FTM2_CH4 | FTM Channel] | PTD14: [FTM2_CH5 | FTM Channel] | PTE11: [FTM2_CH5 | FTM Channel] | PTC12: [FTM2_CH6 | FTM Channel] | PTE15: [FTM2_CH6 | FTM Channel] | PTC13: [FTM2_CH7 | FTM Channel] | PTE16: [FTM2_CH7 | FTM Channel] | PTA2: [FTM3_CH0 | FTM Channel] | PTB8: [FTM3_CH0 | FTM Channel] | PTA3: [FTM3_CH1 | FTM Channel] | PTB9: [FTM3_CH1 | FTM Channel] | PTB10: [FTM3_CH2 | FTM Channel] | PTC6: [FTM3_CH2 | FTM Channel] | PTB11: [FTM3_CH3 | FTM Channel] | PTC7: [FTM3_CH3 | FTM Channel] | PTC10: [FTM3_CH4 | FTM Channel] | PTD2: [FTM3_CH4 | FTM Channel] | PTC11: [FTM3_CH5 | FTM Channel] | PTD3: [FTM3_CH5 | FTM Channel] | PTC12: [FTM3_CH6 | FTM Channel] | PTE2: [FTM3_CH6 | FTM Channel] | PTC13: [FTM3_CH7 | FTM Channel] | PTE6: [FTM3_CH7 | FTM Channel] | PTD15: [FTM0_CH0 | FTM Channel] | PTB13: [FTM0_CH1 | FTM Channel] | PTC1: [FTM0_CH1 | FTM Channel] | PTD16: [FTM0_CH1 | FTM Channel] | PTC2: [FTM0_CH2 | FTM Channel] | PTD0: [FTM0_CH2 | FTM Channel] | PTC3: [FTM0_CH3 | FTM Channel] | PTD1: [FTM0_CH3 | FTM Channel] | PTB4: [FTM0_CH4 | FTM Channel] | PTB5: [FTM0_CH5 | FTM Channel] | PTE8: [FTM0_CH6 | FTM Channel] | PTE9: [FTM0_CH7 | FTM Channel] | PTB2: [FTM1_CH0 | FTM Channel] | PTC4: [FTM1_CH0 | FTM Channel] | PTA1: [FTM1_CH1 | FTM Channel] | PTB3: [FTM1_CH1 | FTM Channel] | PTC14: [FTM1_CH2 | FTM Channel] | PTC15: [FTM1_CH3 | FTM Channel] | PTA10: [FTM1_CH4 | FTM Channel] | PTA11: [FTM1_CH5 | FTM Channel] | PTA12: [FTM1_CH6 | FTM Channel] | PTA13: [FTM1_CH7 | FTM Channel] | PTC1: [FTM1_CH7 | FTM Channel] | PTC5: [FTM2_CH0 | FTM Channel] | PTD0: [FTM2_CH0 | FTM Channel] | PTD10: [FTM2_CH0 | FTM Channel] | PTA0: [FTM2_CH1 | FTM Channel] | PTD1: [FTM2_CH1 | FTM Channel] | PTD11: [FTM2_CH1 | FTM Channel] | PTD12: [FTM2_CH2 | FTM Channel] | PTE4: [FTM2_CH2 | FTM Channel] | PTD5: [FTM2_CH3 | FTM Channel] | PTE5: [FTM2_CH3 | FTM Channel] | PTD13: [FTM2_CH4 | FTM Channel] | PTE10: [FTM2_CH4 | FTM Channel] | PTD14: [FTM2_CH5 | FTM Channel] | PTE11: [FTM2_CH5 | FTM Channel] | PTC12: [FTM2_CH6 | FTM Channel] | PTE15: [FTM2_CH6 | FTM Channel] | PTC13: [FTM2_CH7 | FTM Channel] | PTE16: [FTM2_CH7 | FTM Channel] | PTA2: [FTM3_CH0 | FTM Channel] | PTB8: [FTM3_CH0 | FTM Channel] | PTA3: [FTM3_CH1 | FTM Channel] | PTB9: [FTM3_CH1 | FTM Channel] | PTB10: [FTM3_CH2 | FTM Channel] | PTC6: [FTM3_CH2 | FTM Channel] | PTB11: [FTM3_CH3 | FTM Channel] | PTC7: [FTM3_CH3 | FTM Channel] | PTC10: [FTM3_CH4 | FTM Channel] | PTD2: [FTM3_CH4 | FTM Channel] | PTC11: [FTM3_CH5 | FTM Channel] | PTD3: [FTM3_CH5 | FTM Channel] | PTC12: [FTM3_CH6 | FTM Channel] | PTE2: [FTM3_CH6 | FTM Channel] | PTC13: [FTM3_CH7 | FTM Channel] | PTE6: [FTM3_CH7 | FTM Channel] | PTE20: [FTM4_CH0 | FTM Channel] | PTE21: [FTM4_CH1 | FTM Channel] | PTC11: [FTM4_CH2 | FTM Channel] | PTE22: [FTM4_CH2 | FTM Channel] | PTE23: [FTM4_CH3 | FTM Channel] | PTC27: [FTM4_CH4 | FTM Channel] | PTE24: [FTM4_CH4 | FTM Channel] | PTB1: [FTM4_CH5 | FTM Channel] | PTE13: [FTM4_CH5 | FTM Channel] | PTE25: [FTM4_CH5 | FTM Channel] | PTB0: [FTM4_CH6 | FTM Channel] | PTC28: [FTM4_CH7 | FTM Channel] | PTA25: [FTM5_CH0 | FTM Channel] | PTC9: [FTM5_CH0 | FTM Channel] | PTA26: [FTM5_CH1 | FTM Channel] | PTC8: [FTM5_CH1 | FTM Channel] | PTA27: [FTM5_CH2 | FTM Channel] | PTC29: [FTM5_CH2 | FTM Channel] | PTA7: [FTM5_CH3 | FTM Channel] | PTA28: [FTM5_CH3 | FTM Channel] | PTA29: [FTM5_CH4 | FTM Channel] | PTC30: [FTM5_CH4 | FTM Channel] | PTA6: [FTM5_CH5 | FTM Channel] | PTA30: [FTM5_CH5 | FTM Channel] | PTA31: [FTM5_CH6 | FTM Channel] | PTC31: [FTM5_CH6 | FTM Channel] | PTB18: [FTM5_CH7 | FTM Channel] | PTD18: [FTM5_CH7 | FTM Channel] | PTD15: [FTM0_CH0 | FTM Channel] | PTB13: [FTM0_CH1 | FTM Channel] | PTC1: [FTM0_CH1 | FTM Channel] | PTD16: [FTM0_CH1 | FTM Channel] | PTC2: [FTM0_CH2 | FTM Channel] | PTD0: [FTM0_CH2 | FTM Channel] | PTC3: [FTM0_CH3 | FTM Channel] | PTD1: [FTM0_CH3 | FTM Channel] | PTB4: [FTM0_CH4 | FTM Channel] | PTB5: [FTM0_CH5 | FTM Channel] | PTE8: [FTM0_CH6 | FTM Channel] | PTE9: [FTM0_CH7 | FTM Channel] | PTB2: [FTM1_CH0 | FTM Channel] | PTC4: [FTM1_CH0 | FTM Channel] | PTA1: [FTM1_CH1 | FTM Channel] | PTB3: [FTM1_CH1 | FTM Channel] | PTC14: [FTM1_CH2 | FTM Channel] | PTC15: [FTM1_CH3 | FTM Channel] | PTA10: [FTM1_CH4 | FTM Channel] | PTA11: [FTM1_CH5 | FTM Channel] | PTA12: [FTM1_CH6 | FTM Channel] | PTA13: [FTM1_CH7 | FTM Channel] | PTC1: [FTM1_CH7 | FTM Channel] | PTC5: [FTM2_CH0 | FTM Channel] | PTD0: [FTM2_CH0 | FTM Channel] | PTD10: [FTM2_CH0 | FTM Channel] | PTA0: [FTM2_CH1 | FTM Channel] | PTD1: [FTM2_CH1 | FTM Channel] | PTD11: [FTM2_CH1 | FTM Channel] | PTD12: [FTM2_CH2 | FTM Channel] | PTE4: [FTM2_CH2 | FTM Channel] | PTD5: [FTM2_CH3 | FTM Channel] | PTE5: [FTM2_CH3 | FTM Channel] | PTD13: [FTM2_CH4 | FTM Channel] | PTE10: [FTM2_CH4 | FTM Channel] | PTD14: [FTM2_CH5 | FTM Channel] | PTE11: [FTM2_CH5 | FTM Channel] | PTC12: [FTM2_CH6 | FTM Channel] | PTE15: [FTM2_CH6 | FTM Channel] | PTC13: [FTM2_CH7 | FTM Channel] | PTE16: [FTM2_CH7 | FTM Channel] | PTA2: [FTM3_CH0 | FTM Channel] | PTB8: [FTM3_CH0 | FTM Channel] | PTA3: [FTM3_CH1 | FTM Channel] | PTB9: [FTM3_CH1 | FTM Channel] | PTB10: [FTM3_CH2 | FTM Channel] | PTC6: [FTM3_CH2 | FTM Channel] | PTB11: [FTM3_CH3 | FTM Channel] | PTC7: [FTM3_CH3 | FTM Channel] | PTC10: [FTM3_CH4 | FTM Channel] | PTD2: [FTM3_CH4 | FTM Channel] | PTC11: [FTM3_CH5 | FTM Channel] | PTD3: [FTM3_CH5 | FTM Channel] | PTC12: [FTM3_CH6 | FTM Channel] | PTE2: [FTM3_CH6 | FTM Channel] | PTC13: [FTM3_CH7 | FTM Channel] | PTE6: [FTM3_CH7 | FTM Channel] | PTE20: [FTM4_CH0 | FTM Channel] | PTE21: [FTM4_CH1 | FTM Channel] | PTC11: [FTM4_CH2 | FTM Channel] | PTE22: [FTM4_CH2 | FTM Channel] | PTE23: [FTM4_CH3 | FTM Channel] | PTC27: [FTM4_CH4 | FTM Channel] | PTE24: [FTM4_CH4 | FTM Channel] | PTB1: [FTM4_CH5 | FTM Channel] | PTE13: [FTM4_CH5 | FTM Channel] | PTE25: [FTM4_CH5 | FTM Channel] | PTB0: [FTM4_CH6 | FTM Channel] | PTC28: [FTM4_CH7 | FTM Channel] | PTA25: [FTM5_CH0 | FTM Channel] | PTC9: [FTM5_CH0 | FTM Channel] | PTA26: [FTM5_CH1 | FTM Channel] | PTC8: [FTM5_CH1 | FTM Channel] | PTA27: [FTM5_CH2 | FTM Channel] | PTC29: [FTM5_CH2 | FTM Channel] | PTA7: [FTM5_CH3 | FTM Channel] | PTA28: [FTM5_CH3 | FTM Channel] | PTA29: [FTM5_CH4 | FTM Channel] | PTC30: [FTM5_CH4 | FTM Channel] | PTA6: [FTM5_CH5 | FTM Channel] | PTA30: [FTM5_CH5 | FTM Channel] | PTA31: [FTM5_CH6 | FTM Channel] | PTC31: [FTM5_CH6 | FTM Channel] | PTB18: [FTM5_CH7 | FTM Channel] | PTD18: [FTM5_CH7 | FTM Channel] | PTA18: [FTM6_CH0 | FTM Channel] | PTB20: [FTM6_CH0 | FTM Channel] | PTD19: [FTM6_CH0 | FTM Channel] | PTB21: [FTM6_CH1 | FTM Channel] | PTD20: [FTM6_CH1 | FTM Channel] | PTB22: [FTM6_CH2 | FTM Channel] | PTD21: [FTM6_CH2 | FTM Channel] | PTB23: [FTM6_CH3 | FTM Channel] | PTD22: [FTM6_CH3 | FTM Channel] | PTB24: [FTM6_CH4 | FTM Channel] | PTD23: [FTM6_CH4 | FTM Channel] | PTB25: [FTM6_CH5 | FTM Channel] | PTD24: [FTM6_CH5 | FTM Channel] | PTB26: [FTM6_CH6 | FTM Channel] | PTD25: [FTM6_CH6 | FTM Channel] | PTB27: [FTM6_CH7 | FTM Channel] | PTD26: [FTM6_CH7 | FTM Channel] | PTB28: [FTM7_CH0 | FTM Channel] | PTD27: [FTM7_CH0 | FTM Channel] | PTB29: [FTM7_CH1 | FTM Channel] | PTD28: [FTM7_CH1 | FTM Channel] | PTB30: [FTM7_CH2 | FTM Channel] | PTD29: [FTM7_CH2 | FTM Channel] | PTB31: [FTM7_CH3 | FTM Channel] | PTD30: [FTM7_CH3 | FTM Channel] | PTC18: [FTM7_CH4 | FTM Channel] | PTD31: [FTM7_CH4 | FTM Channel] | PTC19: [FTM7_CH5 | FTM Channel] | PTE17: [FTM7_CH5 | FTM Channel] | PTC20: [FTM7_CH6 | FTM Channel] | PTE18: [FTM7_CH6 | FTM Channel] | PTC21: [FTM7_CH7 | FTM Channel] | PTE19: [FTM7_CH7 | FTM Channel]
      mask TypeOptions pinPolCh6: Active Low | Active High
      mask TypeOptions pinPolCh7: Active Low | Active High
      mask TypeOptions outputComplem6: Main duplicated | Main inverted
      mask TypeOptions outputLevel6: Low | High
      mask TypeOptions outputLevel7: Low | High
      mask TypeOptions pwmSyncTrg: Software trigger | Hardware trigger
      mask Callback pwmSyncTrg: mbd_s32k_ftm_pwm_config_cbk(gcb, 'ftm_sync_trigger')
      mask TypeOptions pwmSyncHwRouting: TRGMUX_FTM0 | TRGMUX_FTM1 | TRGMUX_FTM2 | TRGMUX_FTM3 | TRGMUX_FTM4 | TRGMUX_FTM5 | TRGMUX_FTM6 | TRGMUX_FTM7
      mask TypeOptions pwmSyncInvert: System Clock | PWM Syncronization
      mask TypeOptions pwmSyncOutControl: System Clock | PWM Syncronization
      mask TypeOptions pwmSyncOutMask: System Clock | PWM Syncronization
      mask TypeOptions pwmSyncCounterInitial: System Clock | PWM Syncronization
      mask TypeOptions pwmSyncPoints: Update now | Wait Loading Points
      mask TypeOptions reloadPriority: 0 | 1 | 2 | 3 | 4 | 5 | 6 | 7 | 8 | 9 | 10 | 11 | 12 | 13 | 14 | 15
      mask Callback pwmFaultProtection: mbd_s32k_ftm_pwm_config_cbk(gcb, 'ftm_disen_fault_pins')
      mask TypeOptions pwmFaultClearing: Fault control disabled | Manual Fault control for even channels | Manual Fault control for all channels | Automatic Fault control for all channels
      mask TypeOptions pwmFaultPinState: Safe Value | Tri-state Value
      mask TypeOptions pwmFaultPriority: 0 | 1 | 2 | 3 | 4 | 5 | 6 | 7 | 8 | 9 | 10 | 11 | 12 | 13 | 14 | 15
      mask Callback fault_disen_0: mbd_s32k_ftm_pwm_config_cbk(gcb, 'ftm_disen_fault_pins')
      mask TypeOptions fault_polarity_0: Active High | Active Low
      mask Callback fault_disen_1: mbd_s32k_ftm_pwm_config_cbk(gcb, 'ftm_disen_fault_pins')
      mask TypeOptions fault_polarity_1: Active high | Active low
      mask Callback fault_disen_2: mbd_s32k_ftm_pwm_config_cbk(gcb, 'ftm_disen_fault_pins')
      mask TypeOptions fault_polarity_2: Active high | Active low
      mask Callback fault_disen_3: mbd_s32k_ftm_pwm_config_cbk(gcb, 'ftm_disen_fault_pins')
      mask TypeOptions fault_polarity_3: Active high | Active low
      mask TypeOptions fault_pin_0: None | PTA7: [FTM0_FLT2 | FTM Fault Input] | PTC8: [FTM1_FLT0 | FTM Fault Input] | PTC9: [FTM1_FLT1 | FTM Fault Input] | PTC16: [FTM1_FLT2 | FTM Fault Input] | PTE3: [FTM0_FLT0 | FTM Fault Input] | PTA6: [FTM0_FLT1 | FTM Fault Input] | PTA7: [FTM0_FLT2 | FTM Fault Input] | PTD4: [FTM0_FLT3 | FTM Fault Input] | PTC8: [FTM1_FLT0 | FTM Fault Input] | PTC9: [FTM1_FLT1 | FTM Fault Input] | PTC16: [FTM1_FLT2 | FTM Fault Input] | PTC17: [FTM1_FLT3 | FTM Fault Input] | PTE3: [FTM0_FLT0 | FTM Fault Input] | PTA6: [FTM0_FLT1 | FTM Fault Input] | PTA7: [FTM0_FLT2 | FTM Fault Input] | PTD4: [FTM0_FLT3 | FTM Fault Input] | PTC8: [FTM1_FLT0 | FTM Fault Input] | PTC9: [FTM1_FLT1 | FTM Fault Input] | PTC16: [FTM1_FLT2 | FTM Fault Input] | PTC17: [FTM1_FLT3 | FTM Fault Input] | PTE3: [FTM2_FLT0 | FTM Fault Input] | PTE13: [FTM2_FLT0 | FTM Fault Input] | PTD5: [FTM2_FLT1 | FTM Fault Input] | PTE14: [FTM2_FLT1 | FTM Fault Input] | PTD6: [FTM2_FLT2 | FTM Fault Input] | PTD8: [FTM2_FLT2 | FTM Fault Input] | PTD7: [FTM2_FLT3 | FTM Fault Input] | PTD9: [FTM2_FLT3 | FTM Fault Input] | PTA17: [FTM3_FLT0 | FTM Fault Input] | PTE7: [FTM3_FLT0 | FTM Fault Input] | PTA14: [FTM3_FLT1 | FTM Fault Input] | PTB13: [FTM3_FLT1 | FTM Fault Input] | PTA9: [FTM3_FLT2 | FTM Fault Input] | PTB12: [FTM3_FLT2 | FTM Fault Input] | PTA8: [FTM3_FLT3 | FTM Fault Input] | PTD4: [FTM3_FLT3 | FTM Fault Input] | PTE3: [FTM0_FLT0 | FTM Fault Input] | PTA6: [FTM0_FLT1 | FTM Fault Input] | PTA7: [FTM0_FLT2 | FTM Fault Input] | PTD4: [FTM0_FLT3 | FTM Fault Input] | PTC8: [FTM1_FLT0 | FTM Fault Input] | PTC9: [FTM1_FLT1 | FTM Fault Input] | PTC16: [FTM1_FLT2 | FTM Fault Input] | PTC17: [FTM1_FLT3 | FTM Fault Input] | PTE3: [FTM2_FLT0 | FTM Fault Input] | PTE13: [FTM2_FLT0 | FTM Fault Input] | PTD5: [FTM2_FLT1 | FTM Fault Input] | PTE14: [FTM2_FLT1 | FTM Fault Input] | PTD6: [FTM2_FLT2 | FTM Fault Input] | PTD8: [FTM2_FLT2 | FTM Fault Input] | PTD7: [FTM2_FLT3 | FTM Fault Input] | PTD9: [FTM2_FLT3 | FTM Fault Input] | PTA17: [FTM3_FLT0 | FTM Fault Input] | PTE7: [FTM3_FLT0 | FTM Fault Input] | PTA14: [FTM3_FLT1 | FTM Fault Input] | PTB13: [FTM3_FLT1 | FTM Fault Input] | PTA9: [FTM3_FLT2 | FTM Fault Input] | PTB12: [FTM3_FLT2 | FTM Fault Input] | PTA8: [FTM3_FLT3 | FTM Fault Input] | PTD4: [FTM3_FLT3 | FTM Fault Input] | PTE3: [FTM0_FLT0 | FTM Fault Input] | PTA6: [FTM0_FLT1 | FTM Fault Input] | PTA7: [FTM0_FLT2 | FTM Fault Input] | PTD4: [FTM0_FLT3 | FTM Fault Input] | PTC8: [FTM1_FLT0 | FTM Fault Input] | PTC9: [FTM1_FLT1 | FTM Fault Input] | PTC16: [FTM1_FLT2 | FTM Fault Input] | PTC17: [FTM1_FLT3 | FTM Fault Input] | PTE3: [FTM2_FLT0 | FTM Fault Input] | PTE13: [FTM2_FLT0 | FTM Fault Input] | PTD5: [FTM2_FLT1 | FTM Fault Input] | PTE14: [FTM2_FLT1 | FTM Fault Input] | PTD6: [FTM2_FLT2 | FTM Fault Input] | PTD8: [FTM2_FLT2 | FTM Fault Input] | PTD7: [FTM2_FLT3 | FTM Fault Input] | PTD9: [FTM2_FLT3 | FTM Fault Input] | PTA17: [FTM3_FLT0 | FTM Fault Input] | PTE7: [FTM3_FLT0 | FTM Fault Input] | PTA14: [FTM3_FLT1 | FTM Fault Input] | PTB13: [FTM3_FLT1 | FTM Fault Input] | PTA9: [FTM3_FLT2 | FTM Fault Input] | PTB12: [FTM3_FLT2 | FTM Fault Input] | PTA8: [FTM3_FLT3 | FTM Fault Input] | PTD4: [FTM3_FLT3 | FTM Fault Input] | PTA9: [FTM4_FLT0 | FTM Fault Input] | PTE16: [FTM4_FLT0 | FTM Fault Input] | PTA8: [FTM4_FLT1 | FTM Fault Input] | PTE15: [FTM4_FLT1 | FTM Fault Input] | PTA17: [FTM5_FLT0 | FTM Fault Input] | PTE12: [FTM5_FLT0 | FTM Fault Input] | PTB17: [FTM5_FLT1 | FTM Fault Input] | PTD17: [FTM5_FLT1 | FTM Fault Input] | PTE3: [FTM0_FLT0 | FTM Fault Input] | PTA6: [FTM0_FLT1 | FTM Fault Input] | PTA7: [FTM0_FLT2 | FTM Fault Input] | PTD4: [FTM0_FLT3 | FTM Fault Input] | PTC8: [FTM1_FLT0 | FTM Fault Input] | PTC9: [FTM1_FLT1 | FTM Fault Input] | PTC16: [FTM1_FLT2 | FTM Fault Input] | PTC17: [FTM1_FLT3 | FTM Fault Input] | PTE3: [FTM2_FLT0 | FTM Fault Input] | PTE13: [FTM2_FLT0 | FTM Fault Input] | PTD5: [FTM2_FLT1 | FTM Fault Input] | PTE14: [FTM2_FLT1 | FTM Fault Input] | PTD6: [FTM2_FLT2 | FTM Fault Input] | PTD8: [FTM2_FLT2 | FTM Fault Input] | PTD7: [FTM2_FLT3 | FTM Fault Input] | PTD9: [FTM2_FLT3 | FTM Fault Input] | PTA17: [FTM3_FLT0 | FTM Fault Input] | PTE7: [FTM3_FLT0 | FTM Fault Input] | PTA14: [FTM3_FLT1 | FTM Fault Input] | PTB13: [FTM3_FLT1 | FTM Fault Input] | PTA9: [FTM3_FLT2 | FTM Fault Input] | PTB12: [FTM3_FLT2 | FTM Fault Input] | PTA8: [FTM3_FLT3 | FTM Fault Input] | PTD4: [FTM3_FLT3 | FTM Fault Input] | PTA9: [FTM4_FLT0 | FTM Fault Input] | PTE16: [FTM4_FLT0 | FTM Fault Input] | PTA8: [FTM4_FLT1 | FTM Fault Input] | PTE15: [FTM4_FLT1 | FTM Fault Input] | PTA17: [FTM5_FLT0 | FTM Fault Input] | PTE12: [FTM5_FLT0 | FTM Fault Input] | PTB17: [FTM5_FLT1 | FTM Fault Input] | PTD17: [FTM5_FLT1 | FTM Fault Input] | PTB13: [FTM6_FLT0 | FTM Fault Input] | PTD31: [FTM6_FLT0 | FTM Fault Input] | PTB12: [FTM6_FLT1 | FTM Fault Input] | PTD30: [FTM6_FLT1 | FTM Fault Input] | PTA15: [FTM7_FLT0 | FTM Fault Input] | PTC21: [FTM7_FLT0 | FTM Fault Input] | PTC22: [FTM7_FLT1 | FTM Fault Input] | PTE6: [FTM7_FLT1 | FTM Fault Input]
      mask TypeOptions fault_pin_1: None | PTA7: [FTM0_FLT2 | FTM Fault Input] | PTC8: [FTM1_FLT0 | FTM Fault Input] | PTC9: [FTM1_FLT1 | FTM Fault Input] | PTC16: [FTM1_FLT2 | FTM Fault Input] | PTE3: [FTM0_FLT0 | FTM Fault Input] | PTA6: [FTM0_FLT1 | FTM Fault Input] | PTA7: [FTM0_FLT2 | FTM Fault Input] | PTD4: [FTM0_FLT3 | FTM Fault Input] | PTC8: [FTM1_FLT0 | FTM Fault Input] | PTC9: [FTM1_FLT1 | FTM Fault Input] | PTC16: [FTM1_FLT2 | FTM Fault Input] | PTC17: [FTM1_FLT3 | FTM Fault Input] | PTE3: [FTM0_FLT0 | FTM Fault Input] | PTA6: [FTM0_FLT1 | FTM Fault Input] | PTA7: [FTM0_FLT2 | FTM Fault Input] | PTD4: [FTM0_FLT3 | FTM Fault Input] | PTC8: [FTM1_FLT0 | FTM Fault Input] | PTC9: [FTM1_FLT1 | FTM Fault Input] | PTC16: [FTM1_FLT2 | FTM Fault Input] | PTC17: [FTM1_FLT3 | FTM Fault Input] | PTE3: [FTM2_FLT0 | FTM Fault Input] | PTE13: [FTM2_FLT0 | FTM Fault Input] | PTD5: [FTM2_FLT1 | FTM Fault Input] | PTE14: [FTM2_FLT1 | FTM Fault Input] | PTD6: [FTM2_FLT2 | FTM Fault Input] | PTD8: [FTM2_FLT2 | FTM Fault Input] | PTD7: [FTM2_FLT3 | FTM Fault Input] | PTD9: [FTM2_FLT3 | FTM Fault Input] | PTA17: [FTM3_FLT0 | FTM Fault Input] | PTE7: [FTM3_FLT0 | FTM Fault Input] | PTA14: [FTM3_FLT1 | FTM Fault Input] | PTB13: [FTM3_FLT1 | FTM Fault Input] | PTA9: [FTM3_FLT2 | FTM Fault Input] | PTB12: [FTM3_FLT2 | FTM Fault Input] | PTA8: [FTM3_FLT3 | FTM Fault Input] | PTD4: [FTM3_FLT3 | FTM Fault Input] | PTE3: [FTM0_FLT0 | FTM Fault Input] | PTA6: [FTM0_FLT1 | FTM Fault Input] | PTA7: [FTM0_FLT2 | FTM Fault Input] | PTD4: [FTM0_FLT3 | FTM Fault Input] | PTC8: [FTM1_FLT0 | FTM Fault Input] | PTC9: [FTM1_FLT1 | FTM Fault Input] | PTC16: [FTM1_FLT2 | FTM Fault Input] | PTC17: [FTM1_FLT3 | FTM Fault Input] | PTE3: [FTM2_FLT0 | FTM Fault Input] | PTE13: [FTM2_FLT0 | FTM Fault Input] | PTD5: [FTM2_FLT1 | FTM Fault Input] | PTE14: [FTM2_FLT1 | FTM Fault Input] | PTD6: [FTM2_FLT2 | FTM Fault Input] | PTD8: [FTM2_FLT2 | FTM Fault Input] | PTD7: [FTM2_FLT3 | FTM Fault Input] | PTD9: [FTM2_FLT3 | FTM Fault Input] | PTA17: [FTM3_FLT0 | FTM Fault Input] | PTE7: [FTM3_FLT0 | FTM Fault Input] | PTA14: [FTM3_FLT1 | FTM Fault Input] | PTB13: [FTM3_FLT1 | FTM Fault Input] | PTA9: [FTM3_FLT2 | FTM Fault Input] | PTB12: [FTM3_FLT2 | FTM Fault Input] | PTA8: [FTM3_FLT3 | FTM Fault Input] | PTD4: [FTM3_FLT3 | FTM Fault Input] | PTE3: [FTM0_FLT0 | FTM Fault Input] | PTA6: [FTM0_FLT1 | FTM Fault Input] | PTA7: [FTM0_FLT2 | FTM Fault Input] | PTD4: [FTM0_FLT3 | FTM Fault Input] | PTC8: [FTM1_FLT0 | FTM Fault Input] | PTC9: [FTM1_FLT1 | FTM Fault Input] | PTC16: [FTM1_FLT2 | FTM Fault Input] | PTC17: [FTM1_FLT3 | FTM Fault Input] | PTE3: [FTM2_FLT0 | FTM Fault Input] | PTE13: [FTM2_FLT0 | FTM Fault Input] | PTD5: [FTM2_FLT1 | FTM Fault Input] | PTE14: [FTM2_FLT1 | FTM Fault Input] | PTD6: [FTM2_FLT2 | FTM Fault Input] | PTD8: [FTM2_FLT2 | FTM Fault Input] | PTD7: [FTM2_FLT3 | FTM Fault Input] | PTD9: [FTM2_FLT3 | FTM Fault Input] | PTA17: [FTM3_FLT0 | FTM Fault Input] | PTE7: [FTM3_FLT0 | FTM Fault Input] | PTA14: [FTM3_FLT1 | FTM Fault Input] | PTB13: [FTM3_FLT1 | FTM Fault Input] | PTA9: [FTM3_FLT2 | FTM Fault Input] | PTB12: [FTM3_FLT2 | FTM Fault Input] | PTA8: [FTM3_FLT3 | FTM Fault Input] | PTD4: [FTM3_FLT3 | FTM Fault Input] | PTA9: [FTM4_FLT0 | FTM Fault Input] | PTE16: [FTM4_FLT0 | FTM Fault Input] | PTA8: [FTM4_FLT1 | FTM Fault Input] | PTE15: [FTM4_FLT1 | FTM Fault Input] | PTA17: [FTM5_FLT0 | FTM Fault Input] | PTE12: [FTM5_FLT0 | FTM Fault Input] | PTB17: [FTM5_FLT1 | FTM Fault Input] | PTD17: [FTM5_FLT1 | FTM Fault Input] | PTE3: [FTM0_FLT0 | FTM Fault Input] | PTA6: [FTM0_FLT1 | FTM Fault Input] | PTA7: [FTM0_FLT2 | FTM Fault Input] | PTD4: [FTM0_FLT3 | FTM Fault Input] | PTC8: [FTM1_FLT0 | FTM Fault Input] | PTC9: [FTM1_FLT1 | FTM Fault Input] | PTC16: [FTM1_FLT2 | FTM Fault Input] | PTC17: [FTM1_FLT3 | FTM Fault Input] | PTE3: [FTM2_FLT0 | FTM Fault Input] | PTE13: [FTM2_FLT0 | FTM Fault Input] | PTD5: [FTM2_FLT1 | FTM Fault Input] | PTE14: [FTM2_FLT1 | FTM Fault Input] | PTD6: [FTM2_FLT2 | FTM Fault Input] | PTD8: [FTM2_FLT2 | FTM Fault Input] | PTD7: [FTM2_FLT3 | FTM Fault Input] | PTD9: [FTM2_FLT3 | FTM Fault Input] | PTA17: [FTM3_FLT0 | FTM Fault Input] | PTE7: [FTM3_FLT0 | FTM Fault Input] | PTA14: [FTM3_FLT1 | FTM Fault Input] | PTB13: [FTM3_FLT1 | FTM Fault Input] | PTA9: [FTM3_FLT2 | FTM Fault Input] | PTB12: [FTM3_FLT2 | FTM Fault Input] | PTA8: [FTM3_FLT3 | FTM Fault Input] | PTD4: [FTM3_FLT3 | FTM Fault Input] | PTA9: [FTM4_FLT0 | FTM Fault Input] | PTE16: [FTM4_FLT0 | FTM Fault Input] | PTA8: [FTM4_FLT1 | FTM Fault Input] | PTE15: [FTM4_FLT1 | FTM Fault Input] | PTA17: [FTM5_FLT0 | FTM Fault Input] | PTE12: [FTM5_FLT0 | FTM Fault Input] | PTB17: [FTM5_FLT1 | FTM Fault Input] | PTD17: [FTM5_FLT1 | FTM Fault Input] | PTB13: [FTM6_FLT0 | FTM Fault Input] | PTD31: [FTM6_FLT0 | FTM Fault Input] | PTB12: [FTM6_FLT1 | FTM Fault Input] | PTD30: [FTM6_FLT1 | FTM Fault Input] | PTA15: [FTM7_FLT0 | FTM Fault Input] | PTC21: [FTM7_FLT0 | FTM Fault Input] | PTC22: [FTM7_FLT1 | FTM Fault Input] | PTE6: [FTM7_FLT1 | FTM Fault Input]
      mask TypeOptions fault_pin_2: None | PTA7: [FTM0_FLT2 | FTM Fault Input] | PTC8: [FTM1_FLT0 | FTM Fault Input] | PTC9: [FTM1_FLT1 | FTM Fault Input] | PTC16: [FTM1_FLT2 | FTM Fault Input] | PTE3: [FTM0_FLT0 | FTM Fault Input] | PTA6: [FTM0_FLT1 | FTM Fault Input] | PTA7: [FTM0_FLT2 | FTM Fault Input] | PTD4: [FTM0_FLT3 | FTM Fault Input] | PTC8: [FTM1_FLT0 | FTM Fault Input] | PTC9: [FTM1_FLT1 | FTM Fault Input] | PTC16: [FTM1_FLT2 | FTM Fault Input] | PTC17: [FTM1_FLT3 | FTM Fault Input] | PTE3: [FTM0_FLT0 | FTM Fault Input] | PTA6: [FTM0_FLT1 | FTM Fault Input] | PTA7: [FTM0_FLT2 | FTM Fault Input] | PTD4: [FTM0_FLT3 | FTM Fault Input] | PTC8: [FTM1_FLT0 | FTM Fault Input] | PTC9: [FTM1_FLT1 | FTM Fault Input] | PTC16: [FTM1_FLT2 | FTM Fault Input] | PTC17: [FTM1_FLT3 | FTM Fault Input] | PTE3: [FTM2_FLT0 | FTM Fault Input] | PTE13: [FTM2_FLT0 | FTM Fault Input] | PTD5: [FTM2_FLT1 | FTM Fault Input] | PTE14: [FTM2_FLT1 | FTM Fault Input] | PTD6: [FTM2_FLT2 | FTM Fault Input] | PTD8: [FTM2_FLT2 | FTM Fault Input] | PTD7: [FTM2_FLT3 | FTM Fault Input] | PTD9: [FTM2_FLT3 | FTM Fault Input] | PTA17: [FTM3_FLT0 | FTM Fault Input] | PTE7: [FTM3_FLT0 | FTM Fault Input] | PTA14: [FTM3_FLT1 | FTM Fault Input] | PTB13: [FTM3_FLT1 | FTM Fault Input] | PTA9: [FTM3_FLT2 | FTM Fault Input] | PTB12: [FTM3_FLT2 | FTM Fault Input] | PTA8: [FTM3_FLT3 | FTM Fault Input] | PTD4: [FTM3_FLT3 | FTM Fault Input] | PTE3: [FTM0_FLT0 | FTM Fault Input] | PTA6: [FTM0_FLT1 | FTM Fault Input] | PTA7: [FTM0_FLT2 | FTM Fault Input] | PTD4: [FTM0_FLT3 | FTM Fault Input] | PTC8: [FTM1_FLT0 | FTM Fault Input] | PTC9: [FTM1_FLT1 | FTM Fault Input] | PTC16: [FTM1_FLT2 | FTM Fault Input] | PTC17: [FTM1_FLT3 | FTM Fault Input] | PTE3: [FTM2_FLT0 | FTM Fault Input] | PTE13: [FTM2_FLT0 | FTM Fault Input] | PTD5: [FTM2_FLT1 | FTM Fault Input] | PTE14: [FTM2_FLT1 | FTM Fault Input] | PTD6: [FTM2_FLT2 | FTM Fault Input] | PTD8: [FTM2_FLT2 | FTM Fault Input] | PTD7: [FTM2_FLT3 | FTM Fault Input] | PTD9: [FTM2_FLT3 | FTM Fault Input] | PTA17: [FTM3_FLT0 | FTM Fault Input] | PTE7: [FTM3_FLT0 | FTM Fault Input] | PTA14: [FTM3_FLT1 | FTM Fault Input] | PTB13: [FTM3_FLT1 | FTM Fault Input] | PTA9: [FTM3_FLT2 | FTM Fault Input] | PTB12: [FTM3_FLT2 | FTM Fault Input] | PTA8: [FTM3_FLT3 | FTM Fault Input] | PTD4: [FTM3_FLT3 | FTM Fault Input] | PTE3: [FTM0_FLT0 | FTM Fault Input] | PTA6: [FTM0_FLT1 | FTM Fault Input] | PTA7: [FTM0_FLT2 | FTM Fault Input] | PTD4: [FTM0_FLT3 | FTM Fault Input] | PTC8: [FTM1_FLT0 | FTM Fault Input] | PTC9: [FTM1_FLT1 | FTM Fault Input] | PTC16: [FTM1_FLT2 | FTM Fault Input] | PTC17: [FTM1_FLT3 | FTM Fault Input] | PTE3: [FTM2_FLT0 | FTM Fault Input] | PTE13: [FTM2_FLT0 | FTM Fault Input] | PTD5: [FTM2_FLT1 | FTM Fault Input] | PTE14: [FTM2_FLT1 | FTM Fault Input] | PTD6: [FTM2_FLT2 | FTM Fault Input] | PTD8: [FTM2_FLT2 | FTM Fault Input] | PTD7: [FTM2_FLT3 | FTM Fault Input] | PTD9: [FTM2_FLT3 | FTM Fault Input] | PTA17: [FTM3_FLT0 | FTM Fault Input] | PTE7: [FTM3_FLT0 | FTM Fault Input] | PTA14: [FTM3_FLT1 | FTM Fault Input] | PTB13: [FTM3_FLT1 | FTM Fault Input] | PTA9: [FTM3_FLT2 | FTM Fault Input] | PTB12: [FTM3_FLT2 | FTM Fault Input] | PTA8: [FTM3_FLT3 | FTM Fault Input] | PTD4: [FTM3_FLT3 | FTM Fault Input] | PTA9: [FTM4_FLT0 | FTM Fault Input] | PTE16: [FTM4_FLT0 | FTM Fault Input] | PTA8: [FTM4_FLT1 | FTM Fault Input] | PTE15: [FTM4_FLT1 | FTM Fault Input] | PTA17: [FTM5_FLT0 | FTM Fault Input] | PTE12: [FTM5_FLT0 | FTM Fault Input] | PTB17: [FTM5_FLT1 | FTM Fault Input] | PTD17: [FTM5_FLT1 | FTM Fault Input] | PTE3: [FTM0_FLT0 | FTM Fault Input] | PTA6: [FTM0_FLT1 | FTM Fault Input] | PTA7: [FTM0_FLT2 | FTM Fault Input] | PTD4: [FTM0_FLT3 | FTM Fault Input] | PTC8: [FTM1_FLT0 | FTM Fault Input] | PTC9: [FTM1_FLT1 | FTM Fault Input] | PTC16: [FTM1_FLT2 | FTM Fault Input] | PTC17: [FTM1_FLT3 | FTM Fault Input] | PTE3: [FTM2_FLT0 | FTM Fault Input] | PTE13: [FTM2_FLT0 | FTM Fault Input] | PTD5: [FTM2_FLT1 | FTM Fault Input] | PTE14: [FTM2_FLT1 | FTM Fault Input] | PTD6: [FTM2_FLT2 | FTM Fault Input] | PTD8: [FTM2_FLT2 | FTM Fault Input] | PTD7: [FTM2_FLT3 | FTM Fault Input] | PTD9: [FTM2_FLT3 | FTM Fault Input] | PTA17: [FTM3_FLT0 | FTM Fault Input] | PTE7: [FTM3_FLT0 | FTM Fault Input] | PTA14: [FTM3_FLT1 | FTM Fault Input] | PTB13: [FTM3_FLT1 | FTM Fault Input] | PTA9: [FTM3_FLT2 | FTM Fault Input] | PTB12: [FTM3_FLT2 | FTM Fault Input] | PTA8: [FTM3_FLT3 | FTM Fault Input] | PTD4: [FTM3_FLT3 | FTM Fault Input] | PTA9: [FTM4_FLT0 | FTM Fault Input] | PTE16: [FTM4_FLT0 | FTM Fault Input] | PTA8: [FTM4_FLT1 | FTM Fault Input] | PTE15: [FTM4_FLT1 | FTM Fault Input] | PTA17: [FTM5_FLT0 | FTM Fault Input] | PTE12: [FTM5_FLT0 | FTM Fault Input] | PTB17: [FTM5_FLT1 | FTM Fault Input] | PTD17: [FTM5_FLT1 | FTM Fault Input] | PTB13: [FTM6_FLT0 | FTM Fault Input] | PTD31: [FTM6_FLT0 | FTM Fault Input] | PTB12: [FTM6_FLT1 | FTM Fault Input] | PTD30: [FTM6_FLT1 | FTM Fault Input] | PTA15: [FTM7_FLT0 | FTM Fault Input] | PTC21: [FTM7_FLT0 | FTM Fault Input] | PTC22: [FTM7_FLT1 | FTM Fault Input] | PTE6: [FTM7_FLT1 | FTM Fault Input]
      mask TypeOptions fault_pin_3: None | PTA7: [FTM0_FLT2 | FTM Fault Input] | PTC8: [FTM1_FLT0 | FTM Fault Input] | PTC9: [FTM1_FLT1 | FTM Fault Input] | PTC16: [FTM1_FLT2 | FTM Fault Input] | PTE3: [FTM0_FLT0 | FTM Fault Input] | PTA6: [FTM0_FLT1 | FTM Fault Input] | PTA7: [FTM0_FLT2 | FTM Fault Input] | PTD4: [FTM0_FLT3 | FTM Fault Input] | PTC8: [FTM1_FLT0 | FTM Fault Input] | PTC9: [FTM1_FLT1 | FTM Fault Input] | PTC16: [FTM1_FLT2 | FTM Fault Input] | PTC17: [FTM1_FLT3 | FTM Fault Input] | PTE3: [FTM0_FLT0 | FTM Fault Input] | PTA6: [FTM0_FLT1 | FTM Fault Input] | PTA7: [FTM0_FLT2 | FTM Fault Input] | PTD4: [FTM0_FLT3 | FTM Fault Input] | PTC8: [FTM1_FLT0 | FTM Fault Input] | PTC9: [FTM1_FLT1 | FTM Fault Input] | PTC16: [FTM1_FLT2 | FTM Fault Input] | PTC17: [FTM1_FLT3 | FTM Fault Input] | PTE3: [FTM2_FLT0 | FTM Fault Input] | PTE13: [FTM2_FLT0 | FTM Fault Input] | PTD5: [FTM2_FLT1 | FTM Fault Input] | PTE14: [FTM2_FLT1 | FTM Fault Input] | PTD6: [FTM2_FLT2 | FTM Fault Input] | PTD8: [FTM2_FLT2 | FTM Fault Input] | PTD7: [FTM2_FLT3 | FTM Fault Input] | PTD9: [FTM2_FLT3 | FTM Fault Input] | PTA17: [FTM3_FLT0 | FTM Fault Input] | PTE7: [FTM3_FLT0 | FTM Fault Input] | PTA14: [FTM3_FLT1 | FTM Fault Input] | PTB13: [FTM3_FLT1 | FTM Fault Input] | PTA9: [FTM3_FLT2 | FTM Fault Input] | PTB12: [FTM3_FLT2 | FTM Fault Input] | PTA8: [FTM3_FLT3 | FTM Fault Input] | PTD4: [FTM3_FLT3 | FTM Fault Input] | PTE3: [FTM0_FLT0 | FTM Fault Input] | PTA6: [FTM0_FLT1 | FTM Fault Input] | PTA7: [FTM0_FLT2 | FTM Fault Input] | PTD4: [FTM0_FLT3 | FTM Fault Input] | PTC8: [FTM1_FLT0 | FTM Fault Input] | PTC9: [FTM1_FLT1 | FTM Fault Input] | PTC16: [FTM1_FLT2 | FTM Fault Input] | PTC17: [FTM1_FLT3 | FTM Fault Input] | PTE3: [FTM2_FLT0 | FTM Fault Input] | PTE13: [FTM2_FLT0 | FTM Fault Input] | PTD5: [FTM2_FLT1 | FTM Fault Input] | PTE14: [FTM2_FLT1 | FTM Fault Input] | PTD6: [FTM2_FLT2 | FTM Fault Input] | PTD8: [FTM2_FLT2 | FTM Fault Input] | PTD7: [FTM2_FLT3 | FTM Fault Input] | PTD9: [FTM2_FLT3 | FTM Fault Input] | PTA17: [FTM3_FLT0 | FTM Fault Input] | PTE7: [FTM3_FLT0 | FTM Fault Input] | PTA14: [FTM3_FLT1 | FTM Fault Input] | PTB13: [FTM3_FLT1 | FTM Fault Input] | PTA9: [FTM3_FLT2 | FTM Fault Input] | PTB12: [FTM3_FLT2 | FTM Fault Input] | PTA8: [FTM3_FLT3 | FTM Fault Input] | PTD4: [FTM3_FLT3 | FTM Fault Input] | PTE3: [FTM0_FLT0 | FTM Fault Input] | PTA6: [FTM0_FLT1 | FTM Fault Input] | PTA7: [FTM0_FLT2 | FTM Fault Input] | PTD4: [FTM0_FLT3 | FTM Fault Input] | PTC8: [FTM1_FLT0 | FTM Fault Input] | PTC9: [FTM1_FLT1 | FTM Fault Input] | PTC16: [FTM1_FLT2 | FTM Fault Input] | PTC17: [FTM1_FLT3 | FTM Fault Input] | PTE3: [FTM2_FLT0 | FTM Fault Input] | PTE13: [FTM2_FLT0 | FTM Fault Input] | PTD5: [FTM2_FLT1 | FTM Fault Input] | PTE14: [FTM2_FLT1 | FTM Fault Input] | PTD6: [FTM2_FLT2 | FTM Fault Input] | PTD8: [FTM2_FLT2 | FTM Fault Input] | PTD7: [FTM2_FLT3 | FTM Fault Input] | PTD9: [FTM2_FLT3 | FTM Fault Input] | PTA17: [FTM3_FLT0 | FTM Fault Input] | PTE7: [FTM3_FLT0 | FTM Fault Input] | PTA14: [FTM3_FLT1 | FTM Fault Input] | PTB13: [FTM3_FLT1 | FTM Fault Input] | PTA9: [FTM3_FLT2 | FTM Fault Input] | PTB12: [FTM3_FLT2 | FTM Fault Input] | PTA8: [FTM3_FLT3 | FTM Fault Input] | PTD4: [FTM3_FLT3 | FTM Fault Input] | PTA9: [FTM4_FLT0 | FTM Fault Input] | PTE16: [FTM4_FLT0 | FTM Fault Input] | PTA8: [FTM4_FLT1 | FTM Fault Input] | PTE15: [FTM4_FLT1 | FTM Fault Input] | PTA17: [FTM5_FLT0 | FTM Fault Input] | PTE12: [FTM5_FLT0 | FTM Fault Input] | PTB17: [FTM5_FLT1 | FTM Fault Input] | PTD17: [FTM5_FLT1 | FTM Fault Input] | PTE3: [FTM0_FLT0 | FTM Fault Input] | PTA6: [FTM0_FLT1 | FTM Fault Input] | PTA7: [FTM0_FLT2 | FTM Fault Input] | PTD4: [FTM0_FLT3 | FTM Fault Input] | PTC8: [FTM1_FLT0 | FTM Fault Input] | PTC9: [FTM1_FLT1 | FTM Fault Input] | PTC16: [FTM1_FLT2 | FTM Fault Input] | PTC17: [FTM1_FLT3 | FTM Fault Input] | PTE3: [FTM2_FLT0 | FTM Fault Input] | PTE13: [FTM2_FLT0 | FTM Fault Input] | PTD5: [FTM2_FLT1 | FTM Fault Input] | PTE14: [FTM2_FLT1 | FTM Fault Input] | PTD6: [FTM2_FLT2 | FTM Fault Input] | PTD8: [FTM2_FLT2 | FTM Fault Input] | PTD7: [FTM2_FLT3 | FTM Fault Input] | PTD9: [FTM2_FLT3 | FTM Fault Input] | PTA17: [FTM3_FLT0 | FTM Fault Input] | PTE7: [FTM3_FLT0 | FTM Fault Input] | PTA14: [FTM3_FLT1 | FTM Fault Input] | PTB13: [FTM3_FLT1 | FTM Fault Input] | PTA9: [FTM3_FLT2 | FTM Fault Input] | PTB12: [FTM3_FLT2 | FTM Fault Input] | PTA8: [FTM3_FLT3 | FTM Fault Input] | PTD4: [FTM3_FLT3 | FTM Fault Input] | PTA9: [FTM4_FLT0 | FTM Fault Input] | PTE16: [FTM4_FLT0 | FTM Fault Input] | PTA8: [FTM4_FLT1 | FTM Fault Input] | PTE15: [FTM4_FLT1 | FTM Fault Input] | PTA17: [FTM5_FLT0 | FTM Fault Input] | PTE12: [FTM5_FLT0 | FTM Fault Input] | PTB17: [FTM5_FLT1 | FTM Fault Input] | PTD17: [FTM5_FLT1 | FTM Fault Input] | PTB13: [FTM6_FLT0 | FTM Fault Input] | PTD31: [FTM6_FLT0 | FTM Fault Input] | PTB12: [FTM6_FLT1 | FTM Fault Input] | PTD30: [FTM6_FLT1 | FTM Fault Input] | PTA15: [FTM7_FLT0 | FTM Fault Input] | PTC21: [FTM7_FLT0 | FTM Fault Input] | PTC22: [FTM7_FLT1 | FTM Fault Input] | PTE6: [FTM7_FLT1 | FTM Fault Input]
      mask DialogControl Container22 Prompt: PWM Channel Pairs
      mask DialogControl ftmFreqSettingsContainer Prompt: PWM Frequency Settings
      mask DialogControl ftmDeadtimeSettingsContainer Prompt: PWM Deadtime Settings
      mask DialogControl dutyCycleContainer Prompt: Duty Cycle Settings
      mask DialogControl pinFtmMsg Prompt: Please select at least one channel pair in order to enable the Output Signals.
      mask DialogControl pinPairBox0 Prompt: PWM output pair 0 - 1
      mask DialogControl pinPairBox2 Prompt: PWM output pair 2 - 3
      mask DialogControl pinPairBox4 Prompt: PWM output pair 4 - 5
      mask DialogControl pinPairBox6 Prompt: PWM output pair 6 - 7
      mask DialogControl Container19 Prompt: Reload Opportunities
      mask Display:
      | image('nxp_logo.png', 'top-right');
      | port_label('input',1,'Duty Cycle Ch 0')
      | port_label('output',1,'Duty Cycle Ch 0')
      | disp(maskStr);
  FTM_PWM_Disable_Enable : S-Function  FunctionName=ftm_s32k_pwm_disen  SFunctionDeploymentMode=off  EnableBusSupport=off  mask(FTM_s32k_pwm_disen){ftmModule=0, action=Disable}
      mask prompts: ftmModule "Module"
      mask help: Disables/Enables the PWM for the selected module.
      mask init:
      | mbd_s32k_ftm_display_modules(gcb);
      | maskStr = ['FTM PWM Enable Disable', newline, newline, ...
      |     'Module : ', get_param(gcb,'ftmModule'), newline, ...
      |     ' Action : ', get_param(gcb,'action') ];
      settings: NameChangeFcn=mbd_s32k_name_check(gcb);
      mask Help: web(fullfile(mbd_s32k_block_help, 'ftm', 'ftm_pwm_disen.html'));
      mask TypeOptions ftmModule: 0 | 1 | 2 | 3 | 4 | 5 | 6 | 7
      mask TypeOptions action: Disable | Enable
      mask Display:
      | image('nxp_logo.png', 'top-right');
      | disp(maskStr);
  FTM_TOF_ISR : S-Function  Priority=1  FunctionName=ftm_s32k_tof_isr  Parameters=ftmModule, isrlevel  SFunctionDeploymentMode=off  EnableBusSupport=off  mask(FTM_s32k_tof_isr_block){ftmModule=0, isrlevel=15, mcuTargetUpdate=0}
      mask prompts: ftmModule "Module"; isrlevel "ISR priority"
      mask help: FTM Timer Overflow interrupt handler
      mask init:
      | mbd_s32k_ftm_display_modules(gcb);
      | mbd_s32k_isr_priority_cbk(gcb, 'isrlevel');
      | maskStr = [ 'FTM Input TOF ISR', newline, newline, ...
      |     'Module : ', get_param(gcb,'ftmModule'), newline, ...
      |     'Interrupt Priority: ', get_param(gcb, 'isrlevel')];
      settings: NameChangeFcn=mbd_s32k_name_check(gcb);
      mask Help: web(fullfile(mbd_s32k_block_help, 'ftm', 'ftm_tof_isr_block.html'));
      mask TypeOptions ftmModule: 0 | 1 | 2 | 3 | 4 | 5 | 6 | 7
      mask Callback ftmModule: mbd_s32k_ftm_display_modules(gcb);
      mask TypeOptions isrlevel: 0 | 1 | 2 | 3 | 4 | 5 | 6 | 7 | 8 | 9 | 10 | 11 | 12 | 13 | 14 | 15
      mask Display:
      | image('nxp_logo.png', 'top-right');
      | disp(maskStr);
      | port_label('output',1,'function');
  Input_Edge_Capture : S-Function  FunctionName=ftm_s32k_input_edge_capture  Parameters=funcParam  SFunctionDeploymentMode=off  EnableBusSupport=off  mask(FTM_s32k_input_edge_capture_block){ftmModule=0, channel=0, e_mode=Rising, counter_reset=off, prescaler=1, filter_en=off, filter_value=0, isrlevel=15, mcuTargetUpdate=on, pinFtmCh=PTD15: [FTM0_CH0 | FTM Channel]}
      mask prompts: ftmModule "Module"; e_mode "Edge-sensitive mode"; counter_reset "Counter reset"; prescaler "Prescale Factor"; filter_en "Filter enable"; filter_value "Input Filter value"; isrlevel "ISR priority"; pinFtmCh "Channel input pin"
      mask help: Input Edge Capture block to get time stamp on the channel input event.
      mask init:
      | mbd_s32k_ftm_display_modules(gcb);
      | mbd_s32k_ftm_edge_cbk(gcb, 'single');
      | mbd_s32k_isr_priority_cbk(gcb, 'isrlevel');
      | 
      | [labels, maskStr] = mbd_s32k_ftm_input_edge_init(gcb);
      | set_param(gcb, 'MaskDisplay', labels);
      | 
      | funcParam = [];
      settings: NameChangeFcn=mbd_s32k_name_check(gcb);
      mask Help: web(fullfile(mbd_s32k_block_help, 'ftm', 'input_edge_capture_input.html'));
      mask TypeOptions ftmModule: 0 | 1 | 2 | 3 | 4 | 5 | 6 | 7
      mask Callback ftmModule:
      | mbd_s32k_ftm_display_modules(gcb);
      | mbd_s32k_ftm_edge_cbk(gcb, 'single');
      mask TypeOptions channel: 0 | 1 | 2 | 3 | 4 | 5 | 6 | 7
      mask Callback channel: mbd_s32k_ftm_edge_cbk(gcb, 'single');
      mask TypeOptions e_mode: Rising | Falling | Rising or Falling
      mask TypeOptions prescaler: 1 | 2 | 4 | 8 | 16 | 32 | 64 | 128
      mask Callback filter_en:
      | vis = get_param(gcb, 'MaskVisibilities');
      | 
      | %show/hide Filter value
      | idx = mbd_s32k_get_param_index(gcb, 'filter_value');
      | if strcmp(get_param(gcb,'filter_en'),'on')==1,
      |      vis{idx} = 'on';
      | elseif strcmp(get_param(gcb,'filter_en'),'off')==1,
      |     vis{idx} = 'off';
      | end
      | 
      | set_param(gcb,'MaskVisibilities',vis);
      mask TypeOptions isrlevel: 0 | 1 | 2 | 3 | 4 | 5 | 6 | 7 | 8 | 9 | 10 | 11 | 12 | 13 | 14 | 15
      mask TypeOptions pinFtmCh: PTD15: [FTM0_CH0 | FTM Channel] | PTB13: [FTM0_CH1 | FTM Channel] | PTC1: [FTM0_CH1 | FTM Channel] | PTD16: [FTM0_CH1 | FTM Channel] | PTC2: [FTM0_CH2 | FTM Channel] | PTD0: [FTM0_CH2 | FTM Channel] | PTC3: [FTM0_CH3 | FTM Channel] | PTD1: [FTM0_CH3 | FTM Channel] | PTB4: [FTM0_CH4 | FTM Channel] | PTB5: [FTM0_CH5 | FTM Channel] | PTE8: [FTM0_CH6 | FTM Channel] | PTE9: [FTM0_CH7 | FTM Channel] | PTB2: [FTM1_CH0 | FTM Channel] | PTC4: [FTM1_CH0 | FTM Channel] | PTA1: [FTM1_CH1 | FTM Channel] | PTB3: [FTM1_CH1 | FTM Channel] | PTC14: [FTM1_CH2 | FTM Channel] | PTC15: [FTM1_CH3 | FTM Channel] | PTA10: [FTM1_CH4 | FTM Channel] | PTA11: [FTM1_CH5 | FTM Channel] | PTA12: [FTM1_CH6 | FTM Channel] | PTA13: [FTM1_CH7 | FTM Channel] | PTC1: [FTM1_CH7 | FTM Channel] | PTD15: [FTM0_CH0 | FTM Channel] | PTB13: [FTM0_CH1 | FTM Channel] | PTC1: [FTM0_CH1 | FTM Channel] | PTD16: [FTM0_CH1 | FTM Channel] | PTC2: [FTM0_CH2 | FTM Channel] | PTD0: [FTM0_CH2 | FTM Channel] | PTC3: [FTM0_CH3 | FTM Channel] | PTD1: [FTM0_CH3 | FTM Channel] | PTB4: [FTM0_CH4 | FTM Channel] | PTB5: [FTM0_CH5 | FTM Channel] | PTE8: [FTM0_CH6 | FTM Channel] | PTE9: [FTM0_CH7 | FTM Channel] | PTB2: [FTM1_CH0 | FTM Channel] | PTC4: [FTM1_CH0 | FTM Channel] | PTA1: [FTM1_CH1 | FTM Channel] | PTB3: [FTM1_CH1 | FTM Channel] | PTC14: [FTM1_CH2 | FTM Channel] | PTC15: [FTM1_CH3 | FTM Channel] | PTA10: [FTM1_CH4 | FTM Channel] | PTA11: [FTM1_CH5 | FTM Channel] | PTA12: [FTM1_CH6 | FTM Channel] | PTA13: [FTM1_CH7 | FTM Channel] | PTC1: [FTM1_CH7 | FTM Channel] | PTD15: [FTM0_CH0 | FTM Channel] | PTB13: [FTM0_CH1 | FTM Channel] | PTC1: [FTM0_CH1 | FTM Channel] | PTD16: [FTM0_CH1 | FTM Channel] | PTC2: [FTM0_CH2 | FTM Channel] | PTD0: [FTM0_CH2 | FTM Channel] | PTC3: [FTM0_CH3 | FTM Channel] | PTD1: [FTM0_CH3 | FTM Channel] | PTB4: [FTM0_CH4 | FTM Channel] | PTB5: [FTM0_CH5 | FTM Channel] | PTE8: [FTM0_CH6 | FTM Channel] | PTE9: [FTM0_CH7 | FTM Channel] | PTB2: [FTM1_CH0 | FTM Channel] | PTC4: [FTM1_CH0 | FTM Channel] | PTA1: [FTM1_CH1 | FTM Channel] | PTB3: [FTM1_CH1 | FTM Channel] | PTC14: [FTM1_CH2 | FTM Channel] | PTC15: [FTM1_CH3 | FTM Channel] | PTA10: [FTM1_CH4 | FTM Channel] | PTA11: [FTM1_CH5 | FTM Channel] | PTA12: [FTM1_CH6 | FTM Channel] | PTA13: [FTM1_CH7 | FTM Channel] | PTC1: [FTM1_CH7 | FTM Channel] | PTC5: [FTM2_CH0 | FTM Channel] | PTD0: [FTM2_CH0 | FTM Channel] | PTD10: [FTM2_CH0 | FTM Channel] | PTA0: [FTM2_CH1 | FTM Channel] | PTD1: [FTM2_CH1 | FTM Channel] | PTD11: [FTM2_CH1 | FTM Channel] | PTD12: [FTM2_CH2 | FTM Channel] | PTE4: [FTM2_CH2 | FTM Channel] | PTD5: [FTM2_CH3 | FTM Channel] | PTE5: [FTM2_CH3 | FTM Channel] | PTD13: [FTM2_CH4 | FTM Channel] | PTE10: [FTM2_CH4 | FTM Channel] | PTD14: [FTM2_CH5 | FTM Channel] | PTE11: [FTM2_CH5 | FTM Channel] | PTC12: [FTM2_CH6 | FTM Channel] | PTE15: [FTM2_CH6 | FTM Channel] | PTC13: [FTM2_CH7 | FTM Channel] | PTE16: [FTM2_CH7 | FTM Channel] | PTA2: [FTM3_CH0 | FTM Channel] | PTB8: [FTM3_CH0 | FTM Channel] | PTA3: [FTM3_CH1 | FTM Channel] | PTB9: [FTM3_CH1 | FTM Channel] | PTB10: [FTM3_CH2 | FTM Channel] | PTC6: [FTM3_CH2 | FTM Channel] | PTB11: [FTM3_CH3 | FTM Channel] | PTC7: [FTM3_CH3 | FTM Channel] | PTC10: [FTM3_CH4 | FTM Channel] | PTD2: [FTM3_CH4 | FTM Channel] | PTC11: [FTM3_CH5 | FTM Channel] | PTD3: [FTM3_CH5 | FTM Channel] | PTC12: [FTM3_CH6 | FTM Channel] | PTE2: [FTM3_CH6 | FTM Channel] | PTC13: [FTM3_CH7 | FTM Channel] | PTE6: [FTM3_CH7 | FTM Channel] | PTD15: [FTM0_CH0 | FTM Channel] | PTB13: [FTM0_CH1 | FTM Channel] | PTC1: [FTM0_CH1 | FTM Channel] | PTD16: [FTM0_CH1 | FTM Channel] | PTC2: [FTM0_CH2 | FTM Channel] | PTD0: [FTM0_CH2 | FTM Channel] | PTC3: [FTM0_CH3 | FTM Channel] | PTD1: [FTM0_CH3 | FTM Channel] | PTB4: [FTM0_CH4 | FTM Channel] | PTB5: [FTM0_CH5 | FTM Channel] | PTE8: [FTM0_CH6 | FTM Channel] | PTE9: [FTM0_CH7 | FTM Channel] | PTB2: [FTM1_CH0 | FTM Channel] | PTC4: [FTM1_CH0 | FTM Channel] | PTA1: [FTM1_CH1 | FTM Channel] | PTB3: [FTM1_CH1 | FTM Channel] | PTC14: [FTM1_CH2 | FTM Channel] | PTC15: [FTM1_CH3 | FTM Channel] | PTA10: [FTM1_CH4 | FTM Channel] | PTA11: [FTM1_CH5 | FTM Channel] | PTA12: [FTM1_CH6 | FTM Channel] | PTA13: [FTM1_CH7 | FTM Channel] | PTC1: [FTM1_CH7 | FTM Channel] | PTC5: [FTM2_CH0 | FTM Channel] | PTD0: [FTM2_CH0 | FTM Channel] | PTD10: [FTM2_CH0 | FTM Channel] | PTA0: [FTM2_CH1 | FTM Channel] | PTD1: [FTM2_CH1 | FTM Channel] | PTD11: [FTM2_CH1 | FTM Channel] | PTD12: [FTM2_CH2 | FTM Channel] | PTE4: [FTM2_CH2 | FTM Channel] | PTD5: [FTM2_CH3 | FTM Channel] | PTE5: [FTM2_CH3 | FTM Channel] | PTD13: [FTM2_CH4 | FTM Channel] | PTE10: [FTM2_CH4 | FTM Channel] | PTD14: [FTM2_CH5 | FTM Channel] | PTE11: [FTM2_CH5 | FTM Channel] | PTC12: [FTM2_CH6 | FTM Channel] | PTE15: [FTM2_CH6 | FTM Channel] | PTC13: [FTM2_CH7 | FTM Channel] | PTE16: [FTM2_CH7 | FTM Channel] | PTA2: [FTM3_CH0 | FTM Channel] | PTB8: [FTM3_CH0 | FTM Channel] | PTA3: [FTM3_CH1 | FTM Channel] | PTB9: [FTM3_CH1 | FTM Channel] | PTB10: [FTM3_CH2 | FTM Channel] | PTC6: [FTM3_CH2 | FTM Channel] | PTB11: [FTM3_CH3 | FTM Channel] | PTC7: [FTM3_CH3 | FTM Channel] | PTC10: [FTM3_CH4 | FTM Channel] | PTD2: [FTM3_CH4 | FTM Channel] | PTC11: [FTM3_CH5 | FTM Channel] | PTD3: [FTM3_CH5 | FTM Channel] | PTC12: [FTM3_CH6 | FTM Channel] | PTE2: [FTM3_CH6 | FTM Channel] | PTC13: [FTM3_CH7 | FTM Channel] | PTE6: [FTM3_CH7 | FTM Channel] | PTD15: [FTM0_CH0 | FTM Channel] | PTB13: [FTM0_CH1 | FTM Channel] | PTC1: [FTM0_CH1 | FTM Channel] | PTD16: [FTM0_CH1 | FTM Channel] | PTC2: [FTM0_CH2 | FTM Channel] | PTD0: [FTM0_CH2 | FTM Channel] | PTC3: [FTM0_CH3 | FTM Channel] | PTD1: [FTM0_CH3 | FTM Channel] | PTB4: [FTM0_CH4 | FTM Channel] | PTB5: [FTM0_CH5 | FTM Channel] | PTE8: [FTM0_CH6 | FTM Channel] | PTE9: [FTM0_CH7 | FTM Channel] | PTB2: [FTM1_CH0 | FTM Channel] | PTC4: [FTM1_CH0 | FTM Channel] | PTA1: [FTM1_CH1 | FTM Channel] | PTB3: [FTM1_CH1 | FTM Channel] | PTC14: [FTM1_CH2 | FTM Channel] | PTC15: [FTM1_CH3 | FTM Channel] | PTA10: [FTM1_CH4 | FTM Channel] | PTA11: [FTM1_CH5 | FTM Channel] | PTA12: [FTM1_CH6 | FTM Channel] | PTA13: [FTM1_CH7 | FTM Channel] | PTC1: [FTM1_CH7 | FTM Channel] | PTC5: [FTM2_CH0 | FTM Channel] | PTD0: [FTM2_CH0 | FTM Channel] | PTD10: [FTM2_CH0 | FTM Channel] | PTA0: [FTM2_CH1 | FTM Channel] | PTD1: [FTM2_CH1 | FTM Channel] | PTD11: [FTM2_CH1 | FTM Channel] | PTD12: [FTM2_CH2 | FTM Channel] | PTE4: [FTM2_CH2 | FTM Channel] | PTD5: [FTM2_CH3 | FTM Channel] | PTE5: [FTM2_CH3 | FTM Channel] | PTD13: [FTM2_CH4 | FTM Channel] | PTE10: [FTM2_CH4 | FTM Channel] | PTD14: [FTM2_CH5 | FTM Channel] | PTE11: [FTM2_CH5 | FTM Channel] | PTC12: [FTM2_CH6 | FTM Channel] | PTE15: [FTM2_CH6 | FTM Channel] | PTC13: [FTM2_CH7 | FTM Channel] | PTE16: [FTM2_CH7 | FTM Channel] | PTA2: [FTM3_CH0 | FTM Channel] | PTB8: [FTM3_CH0 | FTM Channel] | PTA3: [FTM3_CH1 | FTM Channel] | PTB9: [FTM3_CH1 | FTM Channel] | PTB10: [FTM3_CH2 | FTM Channel] | PTC6: [FTM3_CH2 | FTM Channel] | PTB11: [FTM3_CH3 | FTM Channel] | PTC7: [FTM3_CH3 | FTM Channel] | PTC10: [FTM3_CH4 | FTM Channel] | PTD2: [FTM3_CH4 | FTM Channel] | PTC11: [FTM3_CH5 | FTM Channel] | PTD3: [FTM3_CH5 | FTM Channel] | PTC12: [FTM3_CH6 | FTM Channel] | PTE2: [FTM3_CH6 | FTM Channel] | PTC13: [FTM3_CH7 | FTM Channel] | PTE6: [FTM3_CH7 | FTM Channel] | PTE20: [FTM4_CH0 | FTM Channel] | PTE21: [FTM4_CH1 | FTM Channel] | PTC11: [FTM4_CH2 | FTM Channel] | PTE22: [FTM4_CH2 | FTM Channel] | PTE23: [FTM4_CH3 | FTM Channel] | PTC27: [FTM4_CH4 | FTM Channel] | PTE24: [FTM4_CH4 | FTM Channel] | PTB1: [FTM4_CH5 | FTM Channel] | PTE13: [FTM4_CH5 | FTM Channel] | PTE25: [FTM4_CH5 | FTM Channel] | PTB0: [FTM4_CH6 | FTM Channel] | PTC28: [FTM4_CH7 | FTM Channel] | PTA25: [FTM5_CH0 | FTM Channel] | PTC9: [FTM5_CH0 | FTM Channel] | PTA26: [FTM5_CH1 | FTM Channel] | PTC8: [FTM5_CH1 | FTM Channel] | PTA27: [FTM5_CH2 | FTM Channel] | PTC29: [FTM5_CH2 | FTM Channel] | PTA7: [FTM5_CH3 | FTM Channel] | PTA28: [FTM5_CH3 | FTM Channel] | PTA29: [FTM5_CH4 | FTM Channel] | PTC30: [FTM5_CH4 | FTM Channel] | PTA6: [FTM5_CH5 | FTM Channel] | PTA30: [FTM5_CH5 | FTM Channel] | PTA31: [FTM5_CH6 | FTM Channel] | PTC31: [FTM5_CH6 | FTM Channel] | PTB18: [FTM5_CH7 | FTM Channel] | PTD18: [FTM5_CH7 | FTM Channel] | PTD15: [FTM0_CH0 | FTM Channel] | PTB13: [FTM0_CH1 | FTM Channel] | PTC1: [FTM0_CH1 | FTM Channel] | PTD16: [FTM0_CH1 | FTM Channel] | PTC2: [FTM0_CH2 | FTM Channel] | PTD0: [FTM0_CH2 | FTM Channel] | PTC3: [FTM0_CH3 | FTM Channel] | PTD1: [FTM0_CH3 | FTM Channel] | PTB4: [FTM0_CH4 | FTM Channel] | PTB5: [FTM0_CH5 | FTM Channel] | PTE8: [FTM0_CH6 | FTM Channel] | PTE9: [FTM0_CH7 | FTM Channel] | PTB2: [FTM1_CH0 | FTM Channel] | PTC4: [FTM1_CH0 | FTM Channel] | PTA1: [FTM1_CH1 | FTM Channel] | PTB3: [FTM1_CH1 | FTM Channel] | PTC14: [FTM1_CH2 | FTM Channel] | PTC15: [FTM1_CH3 | FTM Channel] | PTA10: [FTM1_CH4 | FTM Channel] | PTA11: [FTM1_CH5 | FTM Channel] | PTA12: [FTM1_CH6 | FTM Channel] | PTA13: [FTM1_CH7 | FTM Channel] | PTC1: [FTM1_CH7 | FTM Channel] | PTC5: [FTM2_CH0 | FTM Channel] | PTD0: [FTM2_CH0 | FTM Channel] | PTD10: [FTM2_CH0 | FTM Channel] | PTA0: [FTM2_CH1 | FTM Channel] | PTD1: [FTM2_CH1 | FTM Channel] | PTD11: [FTM2_CH1 | FTM Channel] | PTD12: [FTM2_CH2 | FTM Channel] | PTE4: [FTM2_CH2 | FTM Channel] | PTD5: [FTM2_CH3 | FTM Channel] | PTE5: [FTM2_CH3 | FTM Channel] | PTD13: [FTM2_CH4 | FTM Channel] | PTE10: [FTM2_CH4 | FTM Channel] | PTD14: [FTM2_CH5 | FTM Channel] | PTE11: [FTM2_CH5 | FTM Channel] | PTC12: [FTM2_CH6 | FTM Channel] | PTE15: [FTM2_CH6 | FTM Channel] | PTC13: [FTM2_CH7 | FTM Channel] | PTE16: [FTM2_CH7 | FTM Channel] | PTA2: [FTM3_CH0 | FTM Channel] | PTB8: [FTM3_CH0 | FTM Channel] | PTA3: [FTM3_CH1 | FTM Channel] | PTB9: [FTM3_CH1 | FTM Channel] | PTB10: [FTM3_CH2 | FTM Channel] | PTC6: [FTM3_CH2 | FTM Channel] | PTB11: [FTM3_CH3 | FTM Channel] | PTC7: [FTM3_CH3 | FTM Channel] | PTC10: [FTM3_CH4 | FTM Channel] | PTD2: [FTM3_CH4 | FTM Channel] | PTC11: [FTM3_CH5 | FTM Channel] | PTD3: [FTM3_CH5 | FTM Channel] | PTC12: [FTM3_CH6 | FTM Channel] | PTE2: [FTM3_CH6 | FTM Channel] | PTC13: [FTM3_CH7 | FTM Channel] | PTE6: [FTM3_CH7 | FTM Channel] | PTE20: [FTM4_CH0 | FTM Channel] | PTE21: [FTM4_CH1 | FTM Channel] | PTC11: [FTM4_CH2 | FTM Channel] | PTE22: [FTM4_CH2 | FTM Channel] | PTE23: [FTM4_CH3 | FTM Channel] | PTC27: [FTM4_CH4 | FTM Channel] | PTE24: [FTM4_CH4 | FTM Channel] | PTB1: [FTM4_CH5 | FTM Channel] | PTE13: [FTM4_CH5 | FTM Channel] | PTE25: [FTM4_CH5 | FTM Channel] | PTB0: [FTM4_CH6 | FTM Channel] | PTC28: [FTM4_CH7 | FTM Channel] | PTA25: [FTM5_CH0 | FTM Channel] | PTC9: [FTM5_CH0 | FTM Channel] | PTA26: [FTM5_CH1 | FTM Channel] | PTC8: [FTM5_CH1 | FTM Channel] | PTA27: [FTM5_CH2 | FTM Channel] | PTC29: [FTM5_CH2 | FTM Channel] | PTA7: [FTM5_CH3 | FTM Channel] | PTA28: [FTM5_CH3 | FTM Channel] | PTA29: [FTM5_CH4 | FTM Channel] | PTC30: [FTM5_CH4 | FTM Channel] | PTA6: [FTM5_CH5 | FTM Channel] | PTA30: [FTM5_CH5 | FTM Channel] | PTA31: [FTM5_CH6 | FTM Channel] | PTC31: [FTM5_CH6 | FTM Channel] | PTB18: [FTM5_CH7 | FTM Channel] | PTD18: [FTM5_CH7 | FTM Channel] | PTA18: [FTM6_CH0 | FTM Channel] | PTB20: [FTM6_CH0 | FTM Channel] | PTD19: [FTM6_CH0 | FTM Channel] | PTB21: [FTM6_CH1 | FTM Channel] | PTD20: [FTM6_CH1 | FTM Channel] | PTB22: [FTM6_CH2 | FTM Channel] | PTD21: [FTM6_CH2 | FTM Channel] | PTB23: [FTM6_CH3 | FTM Channel] | PTD22: [FTM6_CH3 | FTM Channel] | PTB24: [FTM6_CH4 | FTM Channel] | PTD23: [FTM6_CH4 | FTM Channel] | PTB25: [FTM6_CH5 | FTM Channel] | PTD24: [FTM6_CH5 | FTM Channel] | PTB26: [FTM6_CH6 | FTM Channel] | PTD25: [FTM6_CH6 | FTM Channel] | PTB27: [FTM6_CH7 | FTM Channel] | PTD26: [FTM6_CH7 | FTM Channel] | PTB28: [FTM7_CH0 | FTM Channel] | PTD27: [FTM7_CH0 | FTM Channel] | PTB29: [FTM7_CH1 | FTM Channel] | PTD28: [FTM7_CH1 | FTM Channel] | PTB30: [FTM7_CH2 | FTM Channel] | PTD29: [FTM7_CH2 | FTM Channel] | PTB31: [FTM7_CH3 | FTM Channel] | PTD30: [FTM7_CH3 | FTM Channel] | PTC18: [FTM7_CH4 | FTM Channel] | PTD31: [FTM7_CH4 | FTM Channel] | PTC19: [FTM7_CH5 | FTM Channel] | PTE17: [FTM7_CH5 | FTM Channel] | PTC20: [FTM7_CH6 | FTM Channel] | PTE18: [FTM7_CH6 | FTM Channel] | PTC21: [FTM7_CH7 | FTM Channel] | PTE19: [FTM7_CH7 | FTM Channel]
      mask Display:
      | image('nxp_logo.png', 'top-right');
      | port_label('output',1,'Trigger');
      | port_label('output',2,'Time Stamp');
      | disp(maskStr);
  Quadrature_Decoder : S-Function  Priority=1  FunctionName=ftm_s32k_quadrature_decoder  Parameters=funcParams  SFunctionDeploymentMode=off  EnableBusSupport=off  mask(FTM_s32k_qd_block){ftmModule=1, ec_mode=Phase A and Phase B, prescaler=1, cntin=0, mod=65535, phA_filtr_en=off, phA_filter=0, phA_pin=PTA1: [FTM1_QD_PHA | FTM quadrature Decode PhaseA], polA=Normal, phB_filtr_en=off, phB_filter=0, phB_pin=PTB2: [FTM1_QD_PHB | FTM quadrature Decode PhaseB], polB=Normal}
      mask prompts: ftmModule "Module"; ec_mode "Encoding  mode"; prescaler "Prescale Factor"; cntin "Counter Minimum Value"; mod "Counter Maximum Value"; phA_filtr_en "Phase A filter enable"; phA_filter "Phase A filter value"; phA_pin "FTM Phase A input pin"; polA "Phase A Polarity"; phB_filtr_en "Phase B filter enable"; phB_filter "Phase B filter value"; phB_pin "FTM Phase B input pin"; polB "Phase B Polarity"
      mask help: Quadrature Decoder mode uses the input signals phase A and B to control the FTM counter increment and decrement.
      mask init:
      | [labels, maskStr] = mbd_s32k_ftm_qd_init(gcb);
      | set_param(gcb, 'MaskDisplay', labels);
      | 
      | funcParams = [];
      | 
      | mbd_s32k_ftm_display_qd_modules(gcb);
      | mbd_s32k_ftm_qd_display_pins();
      settings: NameChangeFcn=mbd_s32k_name_check(gcb);
      mask Help: web(fullfile(mbd_s32k_block_help, 'ftm', 'quadrature_decoder.html'));
      mask TypeOptions ftmModule: 1 | 2
      mask Callback ftmModule: mbd_s32k_ftm_qd_display_pins();
      mask TypeOptions ec_mode: Phase A and Phase B | Count and Direction
      mask TypeOptions prescaler: 1 | 2 | 4 | 8 | 16 | 32 | 64 | 128
      mask Callback phA_filtr_en:
      | vis = get_param(gcb, 'MaskVisibilities');
      | 
      | % show/hide Filter value
      | idx = mbd_s32k_get_param_index(gcb, 'phA_filter');
      | if strcmp(get_param(gcb, 'phA_filtr_en'), 'on')
      |     vis{idx} = 'on';
      | elseif strcmp(get_param(gcb, 'phA_filtr_en'),'off')
      |     vis{idx} = 'off';
      | end
      | 
      | set_param(gcb, 'MaskVisibilities',vis);
      | clear vis;
      mask TypeOptions phA_pin: PTA1: [FTM1_QD_PHA | FTM quadrature Decode PhaseA] | PTB3: [FTM1_QD_PHA | FTM quadrature Decode PhaseA] | PTC7: [FTM1_QD_PHA | FTM quadrature Decode PhaseA] | PTA1: [FTM1_QD_PHA | FTM quadrature Decode PhaseA] | PTB3: [FTM1_QD_PHA | FTM quadrature Decode PhaseA] | PTC7: [FTM1_QD_PHA | FTM quadrature Decode PhaseA] | PTA1: [FTM1_QD_PHA | FTM quadrature Decode PhaseA] | PTB3: [FTM1_QD_PHA | FTM quadrature Decode PhaseA] | PTC7: [FTM1_QD_PHA | FTM quadrature Decode PhaseA] | PTA0: [FTM2_QD_PHA | FTM quadrature Decode PhaseA] | PTA13: [FTM2_QD_PHA | FTM quadrature Decode PhaseA] | PTD11: [FTM2_QD_PHA | FTM quadrature Decode PhaseA] | PTE5: [FTM2_QD_PHA | FTM quadrature Decode PhaseA] | PTA1: [FTM1_QD_PHA | FTM quadrature Decode PhaseA] | PTB3: [FTM1_QD_PHA | FTM quadrature Decode PhaseA] | PTC7: [FTM1_QD_PHA | FTM quadrature Decode PhaseA] | PTA0: [FTM2_QD_PHA | FTM quadrature Decode PhaseA] | PTA13: [FTM2_QD_PHA | FTM quadrature Decode PhaseA] | PTD11: [FTM2_QD_PHA | FTM quadrature Decode PhaseA] | PTE5: [FTM2_QD_PHA | FTM quadrature Decode PhaseA] | PTA1: [FTM1_QD_PHA | FTM quadrature Decode PhaseA] | PTB3: [FTM1_QD_PHA | FTM quadrature Decode PhaseA] | PTC7: [FTM1_QD_PHA | FTM quadrature Decode PhaseA] | PTA0: [FTM2_QD_PHA | FTM quadrature Decode PhaseA] | PTA13: [FTM2_QD_PHA | FTM quadrature Decode PhaseA] | PTD11: [FTM2_QD_PHA | FTM quadrature Decode PhaseA] | PTE5: [FTM2_QD_PHA | FTM quadrature Decode PhaseA] | PTA1: [FTM1_QD_PHA | FTM quadrature Decode PhaseA] | PTB3: [FTM1_QD_PHA | FTM quadrature Decode PhaseA] | PTC7: [FTM1_QD_PHA | FTM quadrature Decode PhaseA] | PTA0: [FTM2_QD_PHA | FTM quadrature Decode PhaseA] | PTA13: [FTM2_QD_PHA | FTM quadrature Decode PhaseA] | PTD11: [FTM2_QD_PHA | FTM quadrature Decode PhaseA] | PTE5: [FTM2_QD_PHA | FTM quadrature Decode PhaseA]
      mask TypeOptions polA: Normal | Inverted
      mask Callback phB_filtr_en:
      | vis = get_param(gcb, 'MaskVisibilities');
      | 
      | % show/hide Filter value
      | idx = mbd_s32k_get_param_index(gcb, 'phB_filter');
      | if strcmp(get_param(gcb, 'phB_filtr_en'), 'on')
      |     vis{idx} = 'on';
      | elseif strcmp(get_param(gcb, 'phB_filtr_en'), 'off')
      |     vis{idx} = 'off';
      | end
      | 
      | set_param(gcb, 'MaskVisibilities',vis);
      | clear vis;
      mask TypeOptions phB_pin: PTB2: [FTM1_QD_PHB | FTM quadrature Decode PhaseB] | PTC4: [FTM1_QD_PHB | FTM quadrature Decode PhaseB] | PTC6: [FTM1_QD_PHB | FTM quadrature Decode PhaseB] | PTB2: [FTM1_QD_PHB | FTM quadrature Decode PhaseB] | PTC4: [FTM1_QD_PHB | FTM quadrature Decode PhaseB] | PTC6: [FTM1_QD_PHB | FTM quadrature Decode PhaseB] | PTB2: [FTM1_QD_PHB | FTM quadrature Decode PhaseB] | PTC4: [FTM1_QD_PHB | FTM quadrature Decode PhaseB] | PTC6: [FTM1_QD_PHB | FTM quadrature Decode PhaseB] | PTA12: [FTM2_QD_PHB | FTM quadrature Decode PhaseB] | PTC5: [FTM2_QD_PHB | FTM quadrature Decode PhaseB] | PTD10: [FTM2_QD_PHB | FTM quadrature Decode PhaseB] | PTE4: [FTM2_QD_PHB | FTM quadrature Decode PhaseB] | PTB2: [FTM1_QD_PHB | FTM quadrature Decode PhaseB] | PTC4: [FTM1_QD_PHB | FTM quadrature Decode PhaseB] | PTC6: [FTM1_QD_PHB | FTM quadrature Decode PhaseB] | PTA12: [FTM2_QD_PHB | FTM quadrature Decode PhaseB] | PTC5: [FTM2_QD_PHB | FTM quadrature Decode PhaseB] | PTD10: [FTM2_QD_PHB | FTM quadrature Decode PhaseB] | PTE4: [FTM2_QD_PHB | FTM quadrature Decode PhaseB] | PTB2: [FTM1_QD_PHB | FTM quadrature Decode PhaseB] | PTC4: [FTM1_QD_PHB | FTM quadrature Decode PhaseB] | PTC6: [FTM1_QD_PHB | FTM quadrature Decode PhaseB] | PTA12: [FTM2_QD_PHB | FTM quadrature Decode PhaseB] | PTC5: [FTM2_QD_PHB | FTM quadrature Decode PhaseB] | PTD10: [FTM2_QD_PHB | FTM quadrature Decode PhaseB] | PTE4: [FTM2_QD_PHB | FTM quadrature Decode PhaseB] | PTB2: [FTM1_QD_PHB | FTM quadrature Decode PhaseB] | PTC4: [FTM1_QD_PHB | FTM quadrature Decode PhaseB] | PTC6: [FTM1_QD_PHB | FTM quadrature Decode PhaseB] | PTA12: [FTM2_QD_PHB | FTM quadrature Decode PhaseB] | PTC5: [FTM2_QD_PHB | FTM quadrature Decode PhaseB] | PTD10: [FTM2_QD_PHB | FTM quadrature Decode PhaseB] | PTE4: [FTM2_QD_PHB | FTM quadrature Decode PhaseB]
      mask TypeOptions polB: Normal | Inverted
      mask Display:
      | image('nxp_logo.png', 'top-right');
      | port_label('output',1,'FTM Counter');
      | port_label('output',2,'FTM Counter Dir');
      | port_label('output',3,'FTM Overflow');
      | port_label('output',4,'FTM Overflow Dir');
      | disp(maskStr);
  Restart_Dual_Edge_Capture : S-Function  FunctionName=ftm_s32k_restart_dec  Parameters=ftmModule,channel  SFunctionDeploymentMode=off  EnableBusSupport=off  mask(FTM_s32k_dual_edge_restart_block){ftmModule=0, channel=0-1}
      mask prompts: ftmModule "Module"; channel "Channel pair"
      mask help: Restart Dual Edge Capture in One-Shot mode.
      mask init:
      | mbd_s32k_ftm_display_modules(gcb);
      | 
      | maskStr = [  'FTM Dual Edge Capture Restart', newline, newline, ...
      |     'Module : ', get_param(gcb,'ftmModule'), newline, ...
      |     ' Channel pair : ', get_param(gcb,'channel') ];
      settings: NameChangeFcn=mbd_s32k_name_check(gcb);
      mask Help: web(fullfile(mbd_s32k_block_help, 'ftm', 'restart_dual_edge_capture.html'));
      mask TypeOptions ftmModule: 0 | 1 | 2 | 3 | 4 | 5 | 6 | 7
      mask Callback ftmModule: mbd_s32k_ftm_display_modules(gcb);
      mask TypeOptions channel: 0-1 | 2-3 | 4-5 | 6-7
      mask Display:
      | image('nxp_logo.png', 'top-right');
      | disp(maskStr);
